simulink model "w2_warplab_buffers"  (Simulink 7.7)
settings: Solver=VariableStepDiscrete  SolverMode=SingleTasking  StartTime=0.0  StopTime=200000  RelTol=1e-3
InitFcn:
  | w2_warplab_buffers_init
StartFcn:
  | w2_warplab_buffers_init
values from neighbouring files (symbols this model uses):
  NumSamps_Rx_IQ = 2^14    (= 16384)    [w2_warplab_buffers_init.m]
  NumSamps_Rx_RSSI = 2^12    (= 4096)    [w2_warplab_buffers_init.m]
  NumSamps_Tx_IQ = 2^14    (= 16384)    [w2_warplab_buffers_init.m]
undefined symbols (not defined in the file or in its folder): gcbh, xlBlockLoadCallback, xlGetNormalizedPeriod
libraries: xbsIndex_r4 x752
(part 2 of 7)

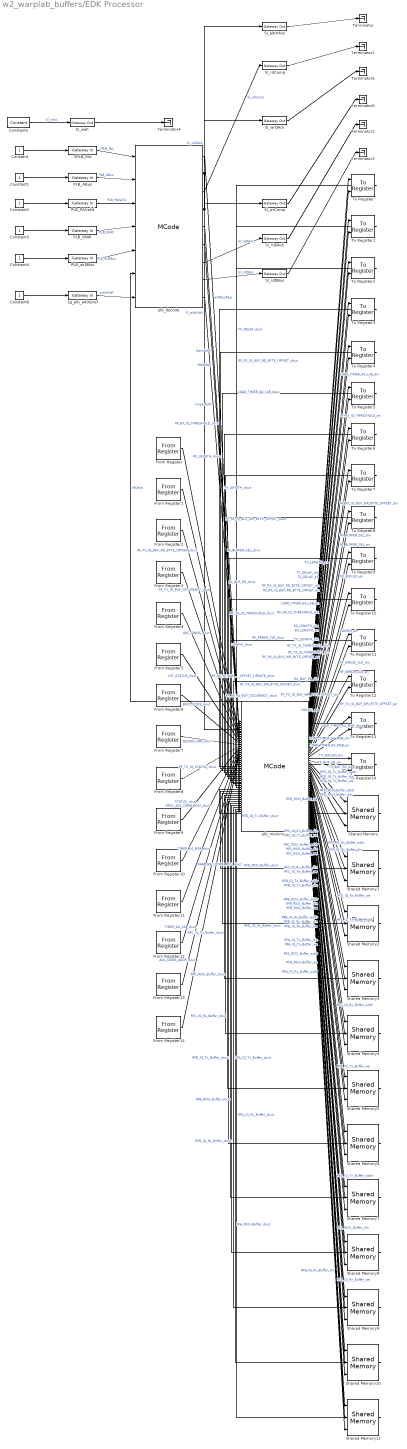
== system w2_warplab_buffers/EDK Processor ==
  Constant{,1..4,6} (6 alike) : Constant
  Constant5 : xbsIndex_r4/Constant  const=0  gui_display_data_type=Fixed-point  arith_type=Unsigned  n_bits=1  bin_pt=0  preci_type=Single  exp_width=8  frac_width=24  explicit_period=on  period=xlGetNormalizedPeriod()  equ=P=C  opselect=C  inp2=PCIN>>17  opr=+  inp1=P  carry=CIN  dbl_ovrd=off  block_type=constant
  From Register : xbsIndex_r4/From Register  shared_memory_name='RF_TX_IQ_BUF_OCCUPANCY'  init=0  period=xlGetNormalizedPeriod()  ownership=Owned and initialized elsewhere  gui_display_data_type=Fixed-point  arith_type=Unsigned  n_bits=32  bin_pt=0  preci_type=Single  dbl_ovrd=off  block_type=fromreg
      settings: AttributesFormatString=<< %<shared_memory_name> >>  infoedit="Register block that reads data to a shared memory register.  Delay of one sample period."
  From Register1 : xbsIndex_r4/From Register  shared_memory_name='RF_TX_IQ_BUF_RD_BYTE_OFFSET'  init=0  period=xlGetNormalizedPeriod()  ownership=Owned and initialized elsewhere  gui_display_data_type=Fixed-point  arith_type=Unsigned  n_bits=32  bin_pt=0  preci_type=Single  dbl_ovrd=off  block_type=fromreg
      settings: AttributesFormatString=<< %<shared_memory_name> >>  infoedit="Register block that reads data to a shared memory register.  Delay of one sample period."
  From Register10 : xbsIndex_r4/From Register  shared_memory_name='RFCD_AGC_DONE_RSSI'  init=0  period=xlGetNormalizedPeriod()  ownership=Owned and initialized elsewhere  gui_display_data_type=Fixed-point  arith_type=Unsigned  n_bits=32  bin_pt=0  preci_type=Single  dbl_ovrd=off  block_type=fromreg
      settings: AttributesFormatString=<< %<shared_memory_name> >>  infoedit="Register block that reads data to a shared memory register.  Delay of one sample period."
  From Register11 : xbsIndex_r4/From Register  shared_memory_name='RFAB_AGC_DONE_RSSI'  init=0  period=xlGetNormalizedPeriod()  ownership=Owned and initialized elsewhere  gui_display_data_type=Fixed-point  arith_type=Unsigned  n_bits=32  bin_pt=0  preci_type=Single  dbl_ovrd=off  block_type=fromreg
      settings: AttributesFormatString=<< %<shared_memory_name> >>  infoedit="Register block that reads data to a shared memory register.  Delay of one sample period."
  From Register12 : xbsIndex_r4/From Register  shared_memory_name='TIMER_64_MSB'  init=0  period=xlGetNormalizedPeriod()  ownership=Owned and initialized elsewhere  gui_display_data_type=Fixed-point  arith_type=Unsigned  n_bits=32  bin_pt=0  preci_type=Single  dbl_ovrd=off  block_type=fromreg
      settings: AttributesFormatString=<< %<shared_memory_name> >>  infoedit="Register block that reads data to a shared memory register.  Delay of one sample period."
  From Register13 : xbsIndex_r4/From Register  shared_memory_name='TIMER_64_LSB'  init=0  period=xlGetNormalizedPeriod()  ownership=Owned and initialized elsewhere  gui_display_data_type=Fixed-point  arith_type=Unsigned  n_bits=32  bin_pt=0  preci_type=Single  dbl_ovrd=off  block_type=fromreg
      settings: AttributesFormatString=<< %<shared_memory_name> >>  infoedit="Register block that reads data to a shared memory register.  Delay of one sample period."
  From Register14 : xbsIndex_r4/From Register  shared_memory_name='AGC_DONE_ADDR'  init=0  period=xlGetNormalizedPeriod()  ownership=Owned and initialized elsewhere  gui_display_data_type=Fixed-point  arith_type=Unsigned  n_bits=32  bin_pt=0  preci_type=Single  dbl_ovrd=off  block_type=fromreg
      settings: AttributesFormatString=<< %<shared_memory_name> >>  infoedit="Register block that reads data to a shared memory register.  Delay of one sample period."
  From Register2 : xbsIndex_r4/From Register  shared_memory_name='AGC_GAINS'  init=0  period=xlGetNormalizedPeriod()  ownership=Owned and initialized elsewhere  gui_display_data_type=Fixed-point  arith_type=Unsigned  n_bits=32  bin_pt=0  preci_type=Single  dbl_ovrd=off  block_type=fromreg
      settings: AttributesFormatString=<< %<shared_memory_name> >>  infoedit="Register block that reads data to a shared memory register.  Delay of one sample period."
  From Register3 : xbsIndex_r4/From Register  shared_memory_name='RF_RX_IQ_BUF_OCCUPANCY'  init=0  period=xlGetNormalizedPeriod()  ownership=Owned and initialized elsewhere  gui_display_data_type=Fixed-point  arith_type=Unsigned  n_bits=32  bin_pt=0  preci_type=Single  dbl_ovrd=off  block_type=fromreg
      settings: AttributesFormatString=<< %<shared_memory_name> >>  infoedit="Register block that reads data to a shared memory register.  Delay of one sample period."
  From Register4 : xbsIndex_r4/From Register  shared_memory_name='RF_RX_IQ_BUF_WR_BYTE_OFFSET_UPDATE'  init=0  period=xlGetNormalizedPeriod()  ownership=Owned and initialized elsewhere  gui_display_data_type=Fixed-point  arith_type=Unsigned  n_bits=32  bin_pt=0  preci_type=Single  dbl_ovrd=off  block_type=fromreg
      settings: AttributesFormatString=<< %<shared_memory_name> >>  infoedit="Register block that reads data to a shared memory register.  Delay of one sample period."
  From Register5 : xbsIndex_r4/From Register  shared_memory_name='INT_STATUS'  init=0  period=xlGetNormalizedPeriod()  ownership=Owned and initialized elsewhere  gui_display_data_type=Fixed-point  arith_type=Unsigned  n_bits=32  bin_pt=0  preci_type=Single  dbl_ovrd=off  block_type=fromreg
      settings: AttributesFormatString=<< %<shared_memory_name> >>  infoedit="Register block that reads data to a shared memory register.  Delay of one sample period."
  From Register6 : xbsIndex_r4/From Register  shared_memory_name='BUFF_SIZES'  init=0  period=xlGetNormalizedPeriod()  ownership=Owned and initialized elsewhere  gui_display_data_type=Fixed-point  arith_type=Unsigned  n_bits=32  bin_pt=0  preci_type=Single  dbl_ovrd=off  block_type=fromreg
      settings: AttributesFormatString=<< %<shared_memory_name> >>  infoedit="Register block that reads data to a shared memory register.  Delay of one sample period."
  From Register7 : xbsIndex_r4/From Register  shared_memory_name='DESIGN_VER'  init=0  period=xlGetNormalizedPeriod()  ownership=Owned and initialized elsewhere  gui_display_data_type=Fixed-point  arith_type=Unsigned  n_bits=32  bin_pt=0  preci_type=Single  dbl_ovrd=off  block_type=fromreg
      settings: AttributesFormatString=<< %<shared_memory_name> >>  infoedit="Register block that reads data to a shared memory register.  Delay of one sample period."
  From Register8 : xbsIndex_r4/From Register  shared_memory_name='RF_TX_IQ_STATUS'  init=0  period=xlGetNormalizedPeriod()  ownership=Owned and initialized elsewhere  gui_display_data_type=Fixed-point  arith_type=Unsigned  n_bits=32  bin_pt=0  preci_type=Single  dbl_ovrd=off  block_type=fromreg
      settings: AttributesFormatString=<< %<shared_memory_name> >>  infoedit="Register block that reads data to a shared memory register.  Delay of one sample period."
  From Register9 : xbsIndex_r4/From Register  shared_memory_name='STATUS'  init=0  period=xlGetNormalizedPeriod()  ownership=Owned and initialized elsewhere  gui_display_data_type=Fixed-point  arith_type=Unsigned  n_bits=32  bin_pt=0  preci_type=Single  dbl_ovrd=off  block_type=fromreg
      settings: AttributesFormatString=<< %<shared_memory_name> >>  infoedit="Register block that reads data to a shared memory register.  Delay of one sample period."
  PLB_ABus : xbsIndex_r4/Gateway In  gui_display_data_type=Fixed-point  arith_type=Unsigned  n_bits=32  bin_pt=0  preci_type=Single  exp_width=8  frac_width=24  quantization="Round  (unbiased: +/- Inf)"  overflow=Saturate  period=xlGetNormalizedPeriod()  dbl_ovrd=off  timing_constraint=None  locs_specified=off  LOCs={}  UseAsADC=off  ADCChannel='1'  inherit_from_input=off  hdl_port=on  block_type=gatewayin
      settings: sginterface={'Xilinx'=>{'jtaghwcosim'=>{'non_memory_mapped_port'=>'PLB_ABus'}},'iopad'=>{'constraint'=>'#'}}
  PLB_PAValid : xbsIndex_r4/Gateway In  gui_display_data_type=Fixed-point  arith_type=Unsigned  n_bits=1  bin_pt=0  preci_type=Single  exp_width=8  frac_width=24  quantization="Round  (unbiased: +/- Inf)"  overflow=Saturate  period=xlGetNormalizedPeriod()  dbl_ovrd=off  timing_constraint=None  locs_specified=off  LOCs={}  UseAsADC=off  ADCChannel='1'  inherit_from_input=off  hdl_port=on  block_type=gatewayin
      settings: sginterface={'Xilinx'=>{'jtaghwcosim'=>{'non_memory_mapped_port'=>'PLB_PAValid'}},'iopad'=>{'constraint'=>'#'}}
  PLB_RNW : xbsIndex_r4/Gateway In  gui_display_data_type=Fixed-point  arith_type=Unsigned  n_bits=1  bin_pt=0  preci_type=Single  exp_width=8  frac_width=24  quantization="Round  (unbiased: +/- Inf)"  overflow=Saturate  period=xlGetNormalizedPeriod()  dbl_ovrd=off  timing_constraint=None  locs_specified=off  LOCs={}  UseAsADC=off  ADCChannel='1'  inherit_from_input=off  hdl_port=on  block_type=gatewayin
      settings: sginterface={'Xilinx'=>{'jtaghwcosim'=>{'non_memory_mapped_port'=>'PLB_RNW'}},'iopad'=>{'constraint'=>'#'}}
  PLB_wrDBus : xbsIndex_r4/Gateway In  gui_display_data_type=Fixed-point  arith_type=Unsigned  n_bits=32  bin_pt=0  preci_type=Single  exp_width=8  frac_width=24  quantization="Round  (unbiased: +/- Inf)"  overflow=Saturate  period=xlGetNormalizedPeriod()  dbl_ovrd=off  timing_constraint=None  locs_specified=off  LOCs={}  UseAsADC=off  ADCChannel='1'  inherit_from_input=off  hdl_port=on  block_type=gatewayin
      settings: sginterface={'Xilinx'=>{'jtaghwcosim'=>{'non_memory_mapped_port'=>'PLB_wrDBus'}},'iopad'=>{'constraint'=>'#'}}
  SPLB_Rst : xbsIndex_r4/Gateway In  gui_display_data_type=Fixed-point  arith_type=Unsigned  n_bits=1  bin_pt=0  preci_type=Single  exp_width=8  frac_width=24  quantization="Round  (unbiased: +/- Inf)"  overflow=Saturate  period=xlGetNormalizedPeriod()  dbl_ovrd=off  timing_constraint=None  locs_specified=off  LOCs={}  UseAsADC=off  ADCChannel='1'  inherit_from_input=off  hdl_port=on  block_type=gatewayin
      settings: sginterface={'Xilinx'=>{'jtaghwcosim'=>{'non_memory_mapped_port'=>'SPLB_Rst'}},'iopad'=>{'constraint'=>'#'}}
  Shared Memory : xbsIndex_r4/Shared Memory  shared_memory_name='RFD_IQ_Tx_Buffer'  depth=16384  ownership=Owned and Initialized Elsewhere  initVector=sin(pi*(0:15)/16)  en=off  mutex=Unprotected  mode=Read and Write  write_mode=Read Before Write  time_out=0  latency=1  explicit_data_type=off  gui_display_data_type=Fixed-point  arith_type=Unsigned  n_bits=32  bin_pt=0  preci_type=Single  implementation=Block RAM  use_rpm=off  block_type=shmem
      settings: AttributesFormatString=<< %<shared_memory_name> >>
  Shared Memory1 : xbsIndex_r4/Shared Memory  shared_memory_name='RFD_RSSI_Buffer'  depth=2048  ownership=Owned and Initialized Elsewhere  initVector=sin(pi*(0:15)/16)  en=off  mutex=Unprotected  mode=Read and Write  write_mode=Read Before Write  time_out=0  latency=1  explicit_data_type=off  gui_display_data_type=Fixed-point  arith_type=Unsigned  n_bits=32  bin_pt=0  preci_type=Single  implementation=Block RAM  use_rpm=off  block_type=shmem
      settings: AttributesFormatString=<< %<shared_memory_name> >>
  Shared Memory10 : xbsIndex_r4/Shared Memory  shared_memory_name='RFA_RSSI_Buffer'  depth=2048  ownership=Owned and Initialized Elsewhere  initVector=sin(pi*(0:15)/16)  en=off  mutex=Unprotected  mode=Read and Write  write_mode=Read Before Write  time_out=0  latency=1  explicit_data_type=off  gui_display_data_type=Fixed-point  arith_type=Unsigned  n_bits=32  bin_pt=0  preci_type=Single  implementation=Block RAM  use_rpm=off  block_type=shmem
      settings: AttributesFormatString=<< %<shared_memory_name> >>
  Shared Memory11 : xbsIndex_r4/Shared Memory  shared_memory_name='RFA_IQ_Rx_Buffer'  depth=16384  ownership=Owned and Initialized Elsewhere  initVector=sin(pi*(0:15)/16)  en=off  mutex=Unprotected  mode=Read and Write  write_mode=Read Before Write  time_out=0  latency=1  explicit_data_type=off  gui_display_data_type=Fixed-point  arith_type=Unsigned  n_bits=32  bin_pt=0  preci_type=Single  implementation=Block RAM  use_rpm=off  block_type=shmem
      settings: AttributesFormatString=<< %<shared_memory_name> >>
  Shared Memory2 : xbsIndex_r4/Shared Memory  shared_memory_name='RFD_IQ_Rx_Buffer'  depth=16384  ownership=Owned and Initialized Elsewhere  initVector=sin(pi*(0:15)/16)  en=off  mutex=Unprotected  mode=Read and Write  write_mode=Read Before Write  time_out=0  latency=1  explicit_data_type=off  gui_display_data_type=Fixed-point  arith_type=Unsigned  n_bits=32  bin_pt=0  preci_type=Single  implementation=Block RAM  use_rpm=off  block_type=shmem
      settings: AttributesFormatString=<< %<shared_memory_name> >>
  Shared Memory3 : xbsIndex_r4/Shared Memory  shared_memory_name='RFC_IQ_Tx_Buffer'  depth=16384  ownership=Owned and Initialized Elsewhere  initVector=sin(pi*(0:15)/16)  en=off  mutex=Unprotected  mode=Read and Write  write_mode=Read Before Write  time_out=0  latency=1  explicit_data_type=off  gui_display_data_type=Fixed-point  arith_type=Unsigned  n_bits=32  bin_pt=0  preci_type=Single  implementation=Block RAM  use_rpm=off  block_type=shmem
      settings: AttributesFormatString=<< %<shared_memory_name> >>
  Shared Memory4 : xbsIndex_r4/Shared Memory  shared_memory_name='RFC_RSSI_Buffer'  depth=2048  ownership=Owned and Initialized Elsewhere  initVector=sin(pi*(0:15)/16)  en=off  mutex=Unprotected  mode=Read and Write  write_mode=Read Before Write  time_out=0  latency=1  explicit_data_type=off  gui_display_data_type=Fixed-point  arith_type=Unsigned  n_bits=32  bin_pt=0  preci_type=Single  implementation=Block RAM  use_rpm=off  block_type=shmem
      settings: AttributesFormatString=<< %<shared_memory_name> >>
  Shared Memory5 : xbsIndex_r4/Shared Memory  shared_memory_name='RFC_IQ_Rx_Buffer'  depth=16384  ownership=Owned and Initialized Elsewhere  initVector=sin(pi*(0:15)/16)  en=off  mutex=Unprotected  mode=Read and Write  write_mode=Read Before Write  time_out=0  latency=1  explicit_data_type=off  gui_display_data_type=Fixed-point  arith_type=Unsigned  n_bits=32  bin_pt=0  preci_type=Single  implementation=Block RAM  use_rpm=off  block_type=shmem
      settings: AttributesFormatString=<< %<shared_memory_name> >>
  Shared Memory6 : xbsIndex_r4/Shared Memory  shared_memory_name='RFB_IQ_Tx_Buffer'  depth=16384  ownership=Owned and Initialized Elsewhere  initVector=sin(pi*(0:15)/16)  en=off  mutex=Unprotected  mode=Read and Write  write_mode=Read Before Write  time_out=0  latency=1  explicit_data_type=off  gui_display_data_type=Fixed-point  arith_type=Unsigned  n_bits=32  bin_pt=0  preci_type=Single  implementation=Block RAM  use_rpm=off  block_type=shmem
      settings: AttributesFormatString=<< %<shared_memory_name> >>
  Shared Memory7 : xbsIndex_r4/Shared Memory  shared_memory_name='RFB_RSSI_Buffer'  depth=2048  ownership=Owned and Initialized Elsewhere  initVector=sin(pi*(0:15)/16)  en=off  mutex=Unprotected  mode=Read and Write  write_mode=Read Before Write  time_out=0  latency=1  explicit_data_type=off  gui_display_data_type=Fixed-point  arith_type=Unsigned  n_bits=32  bin_pt=0  preci_type=Single  implementation=Block RAM  use_rpm=off  block_type=shmem
      settings: AttributesFormatString=<< %<shared_memory_name> >>
  Shared Memory8 : xbsIndex_r4/Shared Memory  shared_memory_name='RFB_IQ_Rx_Buffer'  depth=16384  ownership=Owned and Initialized Elsewhere  initVector=sin(pi*(0:15)/16)  en=off  mutex=Unprotected  mode=Read and Write  write_mode=Read Before Write  time_out=0  latency=1  explicit_data_type=off  gui_display_data_type=Fixed-point  arith_type=Unsigned  n_bits=32  bin_pt=0  preci_type=Single  implementation=Block RAM  use_rpm=off  block_type=shmem
      settings: AttributesFormatString=<< %<shared_memory_name> >>
  Shared Memory9 : xbsIndex_r4/Shared Memory  shared_memory_name='RFA_IQ_Tx_Buffer'  depth=16384  ownership=Owned and Initialized Elsewhere  initVector=sin(pi*(0:15)/16)  en=off  mutex=Unprotected  mode=Read and Write  write_mode=Read Before Write  time_out=0  latency=1  explicit_data_type=off  gui_display_data_type=Fixed-point  arith_type=Unsigned  n_bits=32  bin_pt=0  preci_type=Single  implementation=Block RAM  use_rpm=off  block_type=shmem
      settings: AttributesFormatString=<< %<shared_memory_name> >>
  Sl_addrAck : xbsIndex_r4/Gateway Out  inherit_from_input=off  hdl_port=on  timing_constraint=None  locs_specified=off  LOCs={}  UseAsDAC=off  DACChannel='1'  block_type=gatewayout
      settings: sginterface={'Xilinx'=>{'jtaghwcosim'=>{'non_memory_mapped_port'=>'Sl_addrAck'}},'iopad'=>{'constraint'=>'#'}}
  Sl_rdComp : xbsIndex_r4/Gateway Out  inherit_from_input=off  hdl_port=on  timing_constraint=None  locs_specified=off  LOCs={}  UseAsDAC=off  DACChannel='1'  block_type=gatewayout
      settings: sginterface={'Xilinx'=>{'jtaghwcosim'=>{'non_memory_mapped_port'=>'Sl_rdComp'}},'iopad'=>{'constraint'=>'#'}}
  Sl_rdDAck : xbsIndex_r4/Gateway Out  inherit_from_input=off  hdl_port=on  timing_constraint=None  locs_specified=off  LOCs={}  UseAsDAC=off  DACChannel='1'  block_type=gatewayout
      settings: sginterface={'Xilinx'=>{'jtaghwcosim'=>{'non_memory_mapped_port'=>'Sl_rdDAck'}},'iopad'=>{'constraint'=>'#'}}
  Sl_rdDBus : xbsIndex_r4/Gateway Out  inherit_from_input=off  hdl_port=on  timing_constraint=None  locs_specified=off  LOCs={}  UseAsDAC=off  DACChannel='1'  block_type=gatewayout
      settings: sginterface={'Xilinx'=>{'jtaghwcosim'=>{'non_memory_mapped_port'=>'Sl_rdDBus'}},'iopad'=>{'constraint'=>'#'}}
  Sl_wait : xbsIndex_r4/Gateway Out  inherit_from_input=off  hdl_port=on  timing_constraint=None  locs_specified=off  LOCs={}  UseAsDAC=off  DACChannel='1'  block_type=gatewayout
      settings: sginterface={'Xilinx'=>{'jtaghwcosim'=>{'non_memory_mapped_port'=>'Sl_wait'}},'iopad'=>{'constraint'=>'#'}}
  Sl_wrComp : xbsIndex_r4/Gateway Out  inherit_from_input=off  hdl_port=on  timing_constraint=None  locs_specified=off  LOCs={}  UseAsDAC=off  DACChannel='1'  block_type=gatewayout
      settings: sginterface={'Xilinx'=>{'jtaghwcosim'=>{'non_memory_mapped_port'=>'Sl_wrComp'}},'iopad'=>{'constraint'=>'#'}}
  Sl_wrDAck : xbsIndex_r4/Gateway Out  inherit_from_input=off  hdl_port=on  timing_constraint=None  locs_specified=off  LOCs={}  UseAsDAC=off  DACChannel='1'  block_type=gatewayout
      settings: sginterface={'Xilinx'=>{'jtaghwcosim'=>{'non_memory_mapped_port'=>'Sl_wrDAck'}},'iopad'=>{'constraint'=>'#'}}
  Terminator{,1..6} (7 alike) : Terminator
  To Register : xbsIndex_r4/To Register  shared_memory_name='TX_DELAY'  init=0  ownership=Owned and initialized elsewhere  explicit_data_type=on  gui_display_data_type=Fixed-point  arith_type=Unsigned  n_bits=32  bin_pt=0  preci_type=Single  dbl_ovrd=off  block_type=toreg
      settings: AttributesFormatString=<< %<shared_memory_name> >>  infoedit="Register block that writes data to a shared memory register.  Delay of one sample period."
  To Register1 : xbsIndex_r4/To Register  shared_memory_name='RF_RX_IQ_BUF_RD_BYTE_OFFSET'  init=0  ownership=Owned and initialized elsewhere  explicit_data_type=on  gui_display_data_type=Fixed-point  arith_type=Unsigned  n_bits=32  bin_pt=0  preci_type=Single  dbl_ovrd=off  block_type=toreg
      settings: AttributesFormatString=<< %<shared_memory_name> >>  infoedit="Register block that writes data to a shared memory register.  Delay of one sample period."
  To Register10 : xbsIndex_r4/To Register  shared_memory_name='CONFIG'  init=0  ownership=Owned and initialized elsewhere  explicit_data_type=on  gui_display_data_type=Fixed-point  arith_type=Unsigned  n_bits=32  bin_pt=0  preci_type=Single  dbl_ovrd=off  block_type=toreg
      settings: AttributesFormatString=<< %<shared_memory_name> >>  infoedit="Register block that writes data to a shared memory register.  Delay of one sample period."
  To Register11 : xbsIndex_r4/To Register  shared_memory_name='RF_ERROR_CLR'  init=0  ownership=Owned and initialized elsewhere  explicit_data_type=on  gui_display_data_type=Fixed-point  arith_type=Unsigned  n_bits=9  bin_pt=0  preci_type=Single  dbl_ovrd=off  block_type=toreg
      settings: AttributesFormatString=<< %<shared_memory_name> >>  infoedit="Register block that writes data to a shared memory register.  Delay of one sample period."
  To Register12 : xbsIndex_r4/To Register  shared_memory_name='RF_TX_IQ_BUF_WR_BYTE_OFFSET'  init=0  ownership=Owned and initialized elsewhere  explicit_data_type=on  gui_display_data_type=Fixed-point  arith_type=Unsigned  n_bits=32  bin_pt=0  preci_type=Single  dbl_ovrd=off  block_type=toreg
      settings: AttributesFormatString=<< %<shared_memory_name> >>  infoedit="Register block that writes data to a shared memory register.  Delay of one sample period."
  To Register13 : xbsIndex_r4/To Register  shared_memory_name='LOAD_TIMER_64_MSB'  init=0  ownership=Owned and initialized elsewhere  explicit_data_type=on  gui_display_data_type=Fixed-point  arith_type=Unsigned  n_bits=32  bin_pt=0  preci_type=Single  dbl_ovrd=off  block_type=toreg
      settings: AttributesFormatString=<< %<shared_memory_name> >>  infoedit="Register block that writes data to a shared memory register.  Delay of one sample period."
  To Register14 : xbsIndex_r4/To Register  shared_memory_name='TX_BUF_EN'  init=0  ownership=Owned and initialized elsewhere  explicit_data_type=on  gui_display_data_type=Fixed-point  arith_type=Unsigned  n_bits=32  bin_pt=0  preci_type=Single  dbl_ovrd=off  block_type=toreg
      settings: AttributesFormatString=<< %<shared_memory_name> >>  infoedit="Register block that writes data to a shared memory register.  Delay of one sample period."
  To Register2 : xbsIndex_r4/To Register  shared_memory_name='LOAD_TIMER_64_LSB'  init=0  ownership=Owned and initialized elsewhere  explicit_data_type=on  gui_display_data_type=Fixed-point  arith_type=Unsigned  n_bits=32  bin_pt=0  preci_type=Single  dbl_ovrd=off  block_type=toreg
      settings: AttributesFormatString=<< %<shared_memory_name> >>  infoedit="Register block that writes data to a shared memory register.  Delay of one sample period."
  To Register3 : xbsIndex_r4/To Register  shared_memory_name='RF_RX_IQ_THRESHOLD'  init=0  ownership=Owned and initialized elsewhere  explicit_data_type=on  gui_display_data_type=Fixed-point  arith_type=Unsigned  n_bits=32  bin_pt=0  preci_type=Single  dbl_ovrd=off  block_type=toreg
      settings: AttributesFormatString=<< %<shared_memory_name> >>  infoedit="Register block that writes data to a shared memory register.  Delay of one sample period."
  To Register4 : xbsIndex_r4/To Register  shared_memory_name='RX_LENGTH'  init=0  ownership=Owned and initialized elsewhere  explicit_data_type=on  gui_display_data_type=Fixed-point  arith_type=Unsigned  n_bits=32  bin_pt=0  preci_type=Single  dbl_ovrd=off  block_type=toreg
      settings: AttributesFormatString=<< %<shared_memory_name> >>  infoedit="Register block that writes data to a shared memory register.  Delay of one sample period."
  To Register5 : xbsIndex_r4/To Register  shared_memory_name='TX_LENGTH'  init=0  ownership=Owned and initialized elsewhere  explicit_data_type=on  gui_display_data_type=Fixed-point  arith_type=Unsigned  n_bits=32  bin_pt=0  preci_type=Single  dbl_ovrd=off  block_type=toreg
      settings: AttributesFormatString=<< %<shared_memory_name> >>  infoedit="Register block that writes data to a shared memory register.  Delay of one sample period."
  To Register6 : xbsIndex_r4/To Register  shared_memory_name='RF_RX_IQ_BUF_WR_BYTE_OFFSET'  init=0  ownership=Owned and initialized elsewhere  explicit_data_type=on  gui_display_data_type=Fixed-point  arith_type=Unsigned  n_bits=32  bin_pt=0  preci_type=Single  dbl_ovrd=off  block_type=toreg
      settings: AttributesFormatString=<< %<shared_memory_name> >>  infoedit="Register block that writes data to a shared memory register.  Delay of one sample period."
  To Register7 : xbsIndex_r4/To Register  shared_memory_name='RF_BUFFER_SEL'  init=0  ownership=Owned and initialized elsewhere  explicit_data_type=on  gui_display_data_type=Fixed-point  arith_type=Unsigned  n_bits=32  bin_pt=0  preci_type=Single  dbl_ovrd=off  block_type=toreg
      settings: AttributesFormatString=<< %<shared_memory_name> >>  infoedit="Register block that writes data to a shared memory register.  Delay of one sample period."
  To Register8 : xbsIndex_r4/To Register  shared_memory_name='RX_BUF_EN'  init=0  ownership=Owned and initialized elsewhere  explicit_data_type=on  gui_display_data_type=Fixed-point  arith_type=Unsigned  n_bits=32  bin_pt=0  preci_type=Single  dbl_ovrd=off  block_type=toreg
      settings: AttributesFormatString=<< %<shared_memory_name> >>  infoedit="Register block that writes data to a shared memory register.  Delay of one sample period."
  To Register9 : xbsIndex_r4/To Register  shared_memory_name='RF_TX_IQ_THRESHOLD'  init=0  ownership=Owned and initialized elsewhere  explicit_data_type=on  gui_display_data_type=Fixed-point  arith_type=Unsigned  n_bits=32  bin_pt=0  preci_type=Single  dbl_ovrd=off  block_type=toreg
      settings: AttributesFormatString=<< %<shared_memory_name> >>  infoedit="Register block that writes data to a shared memory register.  Delay of one sample period."
  plb_decode : xbsIndex_r4/MCode  mfname=xlmax  explicit_period=off  period=1  dbl_ovrd=off  enable_stdout=off  enable_debug=off  mfilecontent=|  suppress_output=on  defparams={}  hide_port_list={}  block_type=mcode
      | function [wrDBusReg, addrAck, rdComp, wrDAck, bankAddr, RNWReg, rdDAck, rdDBus, linearAddr] = plb_bus_decode(plbRst, plbABus, plbPAValid, plbRNW, plbWrDBus, rdData, addrPref)
      | 
      | % constant variables (TODO: should pass from outside)
      | ADDRPREF_LEN = 10;
      | BANKADDR_LEN = 2;
      | LINEARADDR_LEN = 18;
      | ABUS_LEN = 32;
      | DBUS_LEN = 32;
      | 
      | % declare and initialize persistent variables
      | % register input bus signals
      | persistent plbRstReg_, plbRstReg_ = xl_state(0, {xlBoolean});
      | persistent plbABusReg_, plbABusReg_ = xl_state(0, {xlUnsigned, ABUS_LEN, 0});
      | persistent plbPAValidReg_, plbPAValidReg_ = xl_state(0, {xlBoolean});
      | persistent plbRNWReg_, plbRNWReg_ = xl_state(0, {xlUnsigned, 1, 0});
      | persistent plbWrDBusReg_, plbWrDBusReg_ = xl_state(0, {xlUnsigned, DBUS_LEN, 0});
      | 
      | % ===== rest of the outputs =====
      | 
      | bankAddr   = xl_slice(plbABusReg_, 2+BANKADDR_LEN+LINEARADDR_LEN-1, 2+LINEARADDR_LEN);
      | linearAddr = xl_slice(plbABusReg_, 2+LINEARADDR_LEN-1, 2);
      | RNWReg = plbRNWReg_;
      | wrDBusReg = plbWrDBusReg_;
      | 
      | % ===== p_select =====
      | 
      | % register PAValid
      | persistent aValidReg, aValidReg = xl_state(0, {xlBoolean});
      | aValidReg = plbPAValidReg_;
      | 
      | % extract and register the address prefix
      | addrPref_in = xl_slice(plbABusReg_, xl_nbits(plbABusReg_)-1, xl_nbits(plbABusReg_)-ADDRPREF_LEN);
      | if addrPref_in == addrPref
      |     ps1 = true;
      | else 
      |     ps1 = false;
      | end 
      | 
      | persistent ps1Reg, ps1Reg = xl_state(0, ps1);
      | ps1Reg = ps1;
      | 
      | ps = xl_and(ps1Reg, aValidReg);
      | 
      | % ===== addrAck =====
      | 
      | % register ps
      | persistent psReg, psReg = xl_state(0, ps);
      | 
      | addrAck = xfix({xlUnsigned, 1, 0}, xl_and(xl_not(plbRstReg_), ps, xl_not(psReg)));
      | 
      | psReg = ps;
      | 
      | % ===== rdComp, rd/wr DAck =====
      |  
      | rdComp1 = xfix({xlUnsigned, 1, 0}, xl_and(addrAck, RNWReg));
      | 
      | NUM_rdCompDelay = 3;
      | persistent rdCompDelay, rdCompDelay = xl_state(zeros(1, NUM_rdCompDelay), rdComp1, NUM_rdCompDelay);
      | rdComp2 = rdCompDelay.back;
      | rdCompDelay.push_front_pop_back(rdComp1);
      | 
      | persistent rdCompReg, rdCompReg = xl_state(0, rdComp1);
      | rdComp = rdCompReg;
      | rdCompReg = rdComp2;
      | 
      | persistent rdDAckReg, rdDAckReg = xl_state(0, rdComp1);
      | rdDAck = rdDAckReg;
      | rdDAckReg = rdComp;
      | 
      | persistent wrDAckReg, wrDAckReg = xl_state(0, addrAck);
      | wrDAck = wrDAckReg;
      | wrDAckReg = xl_and(addrAck, xl_not(RNWReg));
      | 
      | % ===== rdDBus =====
      | 
      | rdSel = xl_or(rdComp2, rdComp);
      | 
      | if rdSel == 1
      |     rdDBus1 = rdData;
      | else
      |     rdDBus1 = 0;
      | end % if
      | 
      | persistent rdDBusReg, rdDBusReg = xl_state(0, rdDBus1);
      | rdDBus = rdDBusReg;
      | rdDBusReg = rdDBus1;
      | 
      | % rdDBus = xl_concat(rdDBus32, rdDBus32);
      | % rdDBus = rdDBus32;
      | 
      | % ===== update the persistent variables =====
      | 
      | plbRstReg_ = plbRst;
      | plbABusReg_ = plbABus;
      | plbPAValidReg_ = plbPAValid;
      | plbRNWReg_ = plbRNW;
      | plbWrDBusReg_ = xl_slice(plbWrDBus, DBUS_LEN-1, 0);
  plb_memmap : xbsIndex_r4/MCode  mfname=xlmax  explicit_period=off  period=1  dbl_ovrd=off  enable_stdout=off  enable_debug=off  mfilecontent=|  suppress_output=on  defparams={}  hide_port_list={}  block_type=mcode
      | function [read_bank_out, sm_TX_DELAY_din, sm_TX_DELAY_en, sm_RF_RX_IQ_BUF_RD_BYTE_OFFSET_din, sm_RF_RX_IQ_BUF_RD_BYTE_OFFSET_en, sm_LOAD_TIMER_64_LSB_din, sm_LOAD_TIMER_64_LSB_en, sm_RF_RX_IQ_THRESHOLD_din, sm_RF_RX_IQ_THRESHOLD_en, sm_RX_LENGTH_din, sm_RX_LENGTH_en, sm_TX_LENGTH_din, sm_TX_LENGTH_en, sm_RF_RX_IQ_BUF_WR_BYTE_OFFSET_din, sm_RF_RX_IQ_BUF_WR_BYTE_OFFSET_en, sm_RF_BUFFER_SEL_din, sm_RF_BUFFER_SEL_en, sm_RX_BUF_EN_din, sm_RX_BUF_EN_en, sm_RF_TX_IQ_THRESHOLD_din, sm_RF_TX_IQ_THRESHOLD_en, sm_CONFIG_din, sm_CONFIG_en, sm_RF_ERROR_CLR_din, sm_RF_ERROR_CLR_en, sm_RF_TX_IQ_BUF_WR_BYTE_OFFSET_din, sm_RF_TX_IQ_BUF_WR_BYTE_OFFSET_en, sm_LOAD_TIMER_64_MSB_din, sm_LOAD_TIMER_64_MSB_en, sm_TX_BUF_EN_din, sm_TX_BUF_EN_en, sm_RFD_IQ_Tx_Buffer_addr, sm_RFD_IQ_Tx_Buffer_din, sm_RFD_IQ_Tx_Buffer_we, sm_RFD_RSSI_Buffer_addr, sm_RFD_RSSI_Buffer_din, sm_RFD_RSSI_Buffer_we, sm_RFD_IQ_Rx_Buffer_addr, sm_RFD_IQ_Rx_Buffer_din, sm_RFD_IQ_Rx_Buffer_we, sm_RFC_IQ_Tx_Buffer_addr, sm_RFC_IQ_Tx_Buffer_din, sm_RFC_IQ_Tx_Buffer_we, sm_RFC_RSSI_Buffer_addr, sm_RFC_RSSI_Buffer_din, sm_RFC_RSSI_Buffer_we, sm_RFC_IQ_Rx_Buffer_addr, sm_RFC_IQ_Rx_Buffer_din, sm_RFC_IQ_Rx_Buffer_we, sm_RFB_IQ_Tx_Buffer_addr, sm_RFB_IQ_Tx_Buffer_din, sm_RFB_IQ_Tx_Buffer_we, sm_RFB_RSSI_Buffer_addr, sm_RFB_RSSI_Buffer_din, sm_RFB_RSSI_Buffer_we, sm_RFB_IQ_Rx_Buffer_addr, sm_RFB_IQ_Rx_Buffer_din, sm_RFB_IQ_Rx_Buffer_we, sm_RFA_IQ_Tx_Buffer_addr, sm_RFA_IQ_Tx_Buffer_din, sm_RFA_IQ_Tx_Buffer_we, sm_RFA_RSSI_Buffer_addr, sm_RFA_RSSI_Buffer_din, sm_RFA_RSSI_Buffer_we, sm_RFA_IQ_Rx_Buffer_addr, sm_RFA_IQ_Rx_Buffer_din, sm_RFA_IQ_Rx_Buffer_we] = plb_memmap(wrDBus, bankAddr, linearAddr, RNWReg, addrAck, sm_RF_TX_IQ_BUF_OCCUPANCY, sm_RF_TX_IQ_BUF_RD_BYTE_OFFSET, sm_AGC_GAINS, sm_RF_RX_IQ_BUF_OCCUPANCY, sm_RF_RX_IQ_BUF_WR_BYTE_OFFSET_UPDATE, sm_INT_STATUS, sm_BUFF_SIZES, sm_DESIGN_VER, sm_RF_TX_IQ_STATUS, sm_STATUS, sm_RFCD_AGC_DONE_RSSI, sm_RFAB_AGC_DONE_RSSI, sm_TIMER_64_MSB, sm_TIMER_64_LSB, sm_AGC_DONE_ADDR, sm_TX_DELAY, sm_RF_RX_IQ_BUF_RD_BYTE_OFFSET, sm_LOAD_TIMER_64_LSB, sm_RF_RX_IQ_THRESHOLD, sm_RX_LENGTH, sm_TX_LENGTH, sm_RF_RX_IQ_BUF_WR_BYTE_OFFSET, sm_RF_BUFFER_SEL, sm_RX_BUF_EN, sm_RF_TX_IQ_THRESHOLD, sm_CONFIG, sm_RF_ERROR_CLR, sm_RF_TX_IQ_BUF_WR_BYTE_OFFSET, sm_LOAD_TIMER_64_MSB, sm_TX_BUF_EN, sm_RFD_IQ_Tx_Buffer, sm_RFD_RSSI_Buffer, sm_RFD_IQ_Rx_Buffer, sm_RFC_IQ_Tx_Buffer, sm_RFC_RSSI_Buffer, sm_RFC_IQ_Rx_Buffer, sm_RFB_IQ_Tx_Buffer, sm_RFB_RSSI_Buffer, sm_RFB_IQ_Rx_Buffer, sm_RFA_IQ_Tx_Buffer, sm_RFA_RSSI_Buffer, sm_RFA_IQ_Rx_Buffer)
      | 
      | 
      | % connvert the input data to UFix_32_0 (the bus data type)
      | % 'From Register' blocks
      | % sm_RF_TX_IQ_BUF_OCCUPANCY_bus = xfix({xlUnsigned, 32, 0}, 0);
      | sm_RF_TX_IQ_BUF_OCCUPANCY_bus = xl_force(sm_RF_TX_IQ_BUF_OCCUPANCY, xlUnsigned, 0);
      | 
      | % sm_RF_TX_IQ_BUF_RD_BYTE_OFFSET_bus = xfix({xlUnsigned, 32, 0}, 0);
      | sm_RF_TX_IQ_BUF_RD_BYTE_OFFSET_bus = xl_force(sm_RF_TX_IQ_BUF_RD_BYTE_OFFSET, xlUnsigned, 0);
      | 
      | % sm_AGC_GAINS_bus = xfix({xlUnsigned, 32, 0}, 0);
      | sm_AGC_GAINS_bus = xl_force(sm_AGC_GAINS, xlUnsigned, 0);
      | 
      | % sm_RF_RX_IQ_BUF_OCCUPANCY_bus = xfix({xlUnsigned, 32, 0}, 0);
      | sm_RF_RX_IQ_BUF_OCCUPANCY_bus = xl_force(sm_RF_RX_IQ_BUF_OCCUPANCY, xlUnsigned, 0);
      | 
      | % sm_RF_RX_IQ_BUF_WR_BYTE_OFFSET_UPDATE_bus = xfix({xlUnsigned, 32, 0}, 0);
      | sm_RF_RX_IQ_BUF_WR_BYTE_OFFSET_UPDATE_bus = xl_force(sm_RF_RX_IQ_BUF_WR_BYTE_OFFSET_UPDATE, xlUnsigned, 0);
      | 
      | % sm_INT_STATUS_bus = xfix({xlUnsigned, 32, 0}, 0);
      | sm_INT_STATUS_bus = xl_force(sm_INT_STATUS, xlUnsigned, 0);
      | 
      | % sm_BUFF_SIZES_bus = xfix({xlUnsigned, 32, 0}, 0);
      | sm_BUFF_SIZES_bus = xl_force(sm_BUFF_SIZES, xlUnsigned, 0);
      | 
      | % sm_DESIGN_VER_bus = xfix({xlUnsigned, 32, 0}, 0);
      | sm_DESIGN_VER_bus = xl_force(sm_DESIGN_VER, xlUnsigned, 0);
      | 
      | % sm_RF_TX_IQ_STATUS_bus = xfix({xlUnsigned, 32, 0}, 0);
      | sm_RF_TX_IQ_STATUS_bus = xl_force(sm_RF_TX_IQ_STATUS, xlUnsigned, 0);
      | 
      | % sm_STATUS_bus = xfix({xlUnsigned, 32, 0}, 0);
      | sm_STATUS_bus = xl_force(sm_STATUS, xlUnsigned, 0);
      | 
      | % sm_RFCD_AGC_DONE_RSSI_bus = xfix({xlUnsigned, 32, 0}, 0);
      | sm_RFCD_AGC_DONE_RSSI_bus = xl_force(sm_RFCD_AGC_DONE_RSSI, xlUnsigned, 0);
      | 
      | % sm_RFAB_AGC_DONE_RSSI_bus = xfix({xlUnsigned, 32, 0}, 0);
      | sm_RFAB_AGC_DONE_RSSI_bus = xl_force(sm_RFAB_AGC_DONE_RSSI, xlUnsigned, 0);
      | 
      | % sm_TIMER_64_MSB_bus = xfix({xlUnsigned, 32, 0}, 0);
      | sm_TIMER_64_MSB_bus = xl_force(sm_TIMER_64_MSB, xlUnsigned, 0);
      | 
      | % sm_TIMER_64_LSB_bus = xfix({xlUnsigned, 32, 0}, 0);
      | sm_TIMER_64_LSB_bus = xl_force(sm_TIMER_64_LSB, xlUnsigned, 0);
      | 
      | % sm_AGC_DONE_ADDR_bus = xfix({xlUnsigned, 32, 0}, 0);
      | sm_AGC_DONE_ADDR_bus = xl_force(sm_AGC_DONE_ADDR, xlUnsigned, 0);
      | 
      | % 'To Register' blocks
      | 
      | % sm_TX_DELAY_dout = xfix({xlUnsigned, 32, 0}, 0);
      | sm_TX_DELAY_dout = xl_force(sm_TX_DELAY, xlUnsigned, 0);
      | 
      | % sm_RF_RX_IQ_BUF_RD_BYTE_OFFSET_dout = xfix({xlUnsigned, 32, 0}, 0);
      | sm_RF_RX_IQ_BUF_RD_BYTE_OFFSET_dout = xl_force(sm_RF_RX_IQ_BUF_RD_BYTE_OFFSET, xlUnsigned, 0);
      | 
      | % sm_LOAD_TIMER_64_LSB_dout = xfix({xlUnsigned, 32, 0}, 0);
      | sm_LOAD_TIMER_64_LSB_dout = xl_force(sm_LOAD_TIMER_64_LSB, xlUnsigned, 0);
      | 
      | % sm_RF_RX_IQ_THRESHOLD_dout = xfix({xlUnsigned, 32, 0}, 0);
      | sm_RF_RX_IQ_THRESHOLD_dout = xl_force(sm_RF_RX_IQ_THRESHOLD, xlUnsigned, 0);
      | 
      | % sm_RX_LENGTH_dout = xfix({xlUnsigned, 32, 0}, 0);
      | sm_RX_LENGTH_dout = xl_force(sm_RX_LENGTH, xlUnsigned, 0);
      | 
      | % sm_TX_LENGTH_dout = xfix({xlUnsigned, 32, 0}, 0);
      | sm_TX_LENGTH_dout = xl_force(sm_TX_LENGTH, xlUnsigned, 0);
      | 
      | % sm_RF_RX_IQ_BUF_WR_BYTE_OFFSET_dout = xfix({xlUnsigned, 32, 0}, 0);
      | sm_RF_RX_IQ_BUF_WR_BYTE_OFFSET_dout = xl_force(sm_RF_RX_IQ_BUF_WR_BYTE_OFFSET, xlUnsigned, 0);
      | 
      | % sm_RF_BUFFER_SEL_dout = xfix({xlUnsigned, 32, 0}, 0);
      | sm_RF_BUFFER_SEL_dout = xl_force(sm_RF_BUFFER_SEL, xlUnsigned, 0);
      | 
      | % sm_RX_BUF_EN_dout = xfix({xlUnsigned, 32, 0}, 0);
      | sm_RX_BUF_EN_dout = xl_force(sm_RX_BUF_EN, xlUnsigned, 0);
      | 
      | % sm_RF_TX_IQ_THRESHOLD_dout = xfix({xlUnsigned, 32, 0}, 0);
      | sm_RF_TX_IQ_THRESHOLD_dout = xl_force(sm_RF_TX_IQ_THRESHOLD, xlUnsigned, 0);
      | 
      | % sm_CONFIG_dout = xfix({xlUnsigned, 32, 0}, 0);
      | sm_CONFIG_dout = xl_force(sm_CONFIG, xlUnsigned, 0);
      | 
      | % sm_RF_ERROR_CLR_dout = xfix({xlUnsigned, 32, 0}, 0);
      | sm_RF_ERROR_CLR_dout = xl_force(sm_RF_ERROR_CLR, xlUnsigned, 0);
      | 
      | % sm_RF_TX_IQ_BUF_WR_BYTE_OFFSET_dout = xfix({xlUnsigned, 32, 0}, 0);
      | sm_RF_TX_IQ_BUF_WR_BYTE_OFFSET_dout = xl_force(sm_RF_TX_IQ_BUF_WR_BYTE_OFFSET, xlUnsigned, 0);
      | 
      | % sm_LOAD_TIMER_64_MSB_dout = xfix({xlUnsigned, 32, 0}, 0);
      | sm_LOAD_TIMER_64_MSB_dout = xl_force(sm_LOAD_TIMER_64_MSB, xlUnsigned, 0);
      | 
      | % sm_TX_BUF_EN_dout = xfix({xlUnsigned, 32, 0}, 0);
      | sm_TX_BUF_EN_dout = xl_force(sm_TX_BUF_EN, xlUnsigned, 0);
      | 
      | 
      | % 'From FIFO' blocks
      | % 'To FIFO' blocks
      | % 'Shared Memory' blocks
      | % RFD_IQ_Tx_Buffer_bus = xfix({xlUnsigned, 32, 0}, 0);
      | sm_RFD_IQ_Tx_Buffer_bus = xl_force(sm_RFD_IQ_Tx_Buffer, xlUnsigned, 0);
      | 
      | % RFD_RSSI_Buffer_bus = xfix({xlUnsigned, 32, 0}, 0);
      | sm_RFD_RSSI_Buffer_bus = xl_force(sm_RFD_RSSI_Buffer, xlUnsigned, 0);
      | 
      | % RFD_IQ_Rx_Buffer_bus = xfix({xlUnsigned, 32, 0}, 0);
      | sm_RFD_IQ_Rx_Buffer_bus = xl_force(sm_RFD_IQ_Rx_Buffer, xlUnsigned, 0);
      | 
      | % RFC_IQ_Tx_Buffer_bus = xfix({xlUnsigned, 32, 0}, 0);
      | sm_RFC_IQ_Tx_Buffer_bus = xl_force(sm_RFC_IQ_Tx_Buffer, xlUnsigned, 0);
      | 
      | % RFC_RSSI_Buffer_bus = xfix({xlUnsigned, 32, 0}, 0);
      | sm_RFC_RSSI_Buffer_bus = xl_force(sm_RFC_RSSI_Buffer, xlUnsigned, 0);
      | 
      | % RFC_IQ_Rx_Buffer_bus = xfix({xlUnsigned, 32, 0}, 0);
      | sm_RFC_IQ_Rx_Buffer_bus = xl_force(sm_RFC_IQ_Rx_Buffer, xlUnsigned, 0);
      | 
      | % RFB_IQ_Tx_Buffer_bus = xfix({xlUnsigned, 32, 0}, 0);
      | sm_RFB_IQ_Tx_Buffer_bus = xl_force(sm_RFB_IQ_Tx_Buffer, xlUnsigned, 0);
      | 
      | % RFB_RSSI_Buffer_bus = xfix({xlUnsigned, 32, 0}, 0);
      | sm_RFB_RSSI_Buffer_bus = xl_force(sm_RFB_RSSI_Buffer, xlUnsigned, 0);
      | 
      | % RFB_IQ_Rx_Buffer_bus = xfix({xlUnsigned, 32, 0}, 0);
      | sm_RFB_IQ_Rx_Buffer_bus = xl_force(sm_RFB_IQ_Rx_Buffer, xlUnsigned, 0);
      | 
      | % RFA_IQ_Tx_Buffer_bus = xfix({xlUnsigned, 32, 0}, 0);
      | sm_RFA_IQ_Tx_Buffer_bus = xl_force(sm_RFA_IQ_Tx_Buffer, xlUnsigned, 0);
      | 
      | % RFA_RSSI_Buffer_bus = xfix({xlUnsigned, 32, 0}, 0);
      | sm_RFA_RSSI_Buffer_bus = xl_force(sm_RFA_RSSI_Buffer, xlUnsigned, 0);
      | 
      | % RFA_IQ_Rx_Buffer_bus = xfix({xlUnsigned, 32, 0}, 0);
      | sm_RFA_IQ_Rx_Buffer_bus = xl_force(sm_RFA_IQ_Rx_Buffer, xlUnsigned, 0);
      | 
      | 
      | % 'dout' ports of 'From Register' blocks
      | 
      | % registered register mux output
      | persistent reg_bank_out_reg; reg_bank_out_reg = xl_state(0, {xlUnsigned, 32, 0});
      | reg_bank_out = reg_bank_out_reg;
      | 
      | if linearAddr == 15
      |     reg_bank_out_reg = sm_RF_TX_IQ_BUF_OCCUPANCY_bus;
      | elseif linearAddr == 16
      |     reg_bank_out_reg = sm_RF_TX_IQ_BUF_RD_BYTE_OFFSET_bus;
      | elseif linearAddr == 17
      |     reg_bank_out_reg = sm_AGC_GAINS_bus;
      | elseif linearAddr == 18
      |     reg_bank_out_reg = sm_RF_RX_IQ_BUF_OCCUPANCY_bus;
      | elseif linearAddr == 19
      |     reg_bank_out_reg = sm_RF_RX_IQ_BUF_WR_BYTE_OFFSET_UPDATE_bus;
      | elseif linearAddr == 20
      |     reg_bank_out_reg = sm_INT_STATUS_bus;
      | elseif linearAddr == 21
      |     reg_bank_out_reg = sm_BUFF_SIZES_bus;
      | elseif linearAddr == 22
      |     reg_bank_out_reg = sm_DESIGN_VER_bus;
      | elseif linearAddr == 23
      |     reg_bank_out_reg = sm_RF_TX_IQ_STATUS_bus;
      | elseif linearAddr == 24
      |     reg_bank_out_reg = sm_STATUS_bus;
      | elseif linearAddr == 25
      |     reg_bank_out_reg = sm_RFCD_AGC_DONE_RSSI_bus;
      | elseif linearAddr == 26
      |     reg_bank_out_reg = sm_RFAB_AGC_DONE_RSSI_bus;
      | elseif linearAddr == 27
      |     reg_bank_out_reg = sm_TIMER_64_MSB_bus;
      | elseif linearAddr == 28
      |     reg_bank_out_reg = sm_TIMER_64_LSB_bus;
      | elseif linearAddr == 29
      |     reg_bank_out_reg = sm_AGC_DONE_ADDR_bus;
      | elseif linearAddr == 0
      |     reg_bank_out_reg = sm_TX_DELAY_dout;
      | elseif linearAddr == 1
      |     reg_bank_out_reg = sm_RF_RX_IQ_BUF_RD_BYTE_OFFSET_dout;
      | elseif linearAddr == 2
      |     reg_bank_out_reg = sm_LOAD_TIMER_64_LSB_dout;
      | elseif linearAddr == 3
      |     reg_bank_out_reg = sm_RF_RX_IQ_THRESHOLD_dout;
      | elseif linearAddr == 4
      |     reg_bank_out_reg = sm_RX_LENGTH_dout;
      | elseif linearAddr == 5
      |     reg_bank_out_reg = sm_TX_LENGTH_dout;
      | elseif linearAddr == 6
      |     reg_bank_out_reg = sm_RF_RX_IQ_BUF_WR_BYTE_OFFSET_dout;
      | elseif linearAddr == 7
      |     reg_bank_out_reg = sm_RF_BUFFER_SEL_dout;
      | elseif linearAddr == 8
      |     reg_bank_out_reg = sm_RX_BUF_EN_dout;
      | elseif linearAddr == 9
      |     reg_bank_out_reg = sm_RF_TX_IQ_THRESHOLD_dout;
      | elseif linearAddr == 10
      |     reg_bank_out_reg = sm_CONFIG_dout;
      | elseif linearAddr == 11
      |     reg_bank_out_reg = sm_RF_ERROR_CLR_dout;
      | elseif linearAddr == 12
      |     reg_bank_out_reg = sm_RF_TX_IQ_BUF_WR_BYTE_OFFSET_dout;
      | elseif linearAddr == 13
      |     reg_bank_out_reg = sm_LOAD_TIMER_64_MSB_dout;
      | elseif linearAddr == 14
      |     reg_bank_out_reg = sm_TX_BUF_EN_dout;
      | 
      | end
      | 
      | 
      | % 'From FIFO' and 'To FIFO' blocks
      | 
      | 
      | 
      | 
      | 
      | opCode = xl_concat(addrAck, RNWReg, bankAddr, linearAddr);
      | 
      | % 'Shared Memory' blocks
      | 
      | sm_RFD_IQ_Tx_Buffer_sel_value = xl_concat(xl_slice(linearAddr, ...
      |                                         xl_nbits(linearAddr) - 1, ...
      |                                         14) ...
      |                                     );
      | if sm_RFD_IQ_Tx_Buffer_sel_value == xfix({xlUnsigned, ...
      |                                         xl_nbits(linearAddr) - 14, ...
      |                                         0}, ...
      |                                         0);
      |     sm_RFD_IQ_Tx_Buffer_sel = true;
      | else
      |     sm_RFD_IQ_Tx_Buffer_sel = false;
      | end
      | sm_RFD_RSSI_Buffer_sel_value = xl_concat(xl_slice(linearAddr, ...
      |                                         xl_nbits(linearAddr) - 1, ...
      |                                         11) ...
      |                                     );
      | if sm_RFD_RSSI_Buffer_sel_value == xfix({xlUnsigned, ...
      |                                         xl_nbits(linearAddr) - 11, ...
      |                                         0}, ...
      |                                         64);
      |     sm_RFD_RSSI_Buffer_sel = true;
      | else
      |     sm_RFD_RSSI_Buffer_sel = false;
      | end
      | sm_RFD_IQ_Rx_Buffer_sel_value = xl_concat(xl_slice(linearAddr, ...
      |                                         xl_nbits(linearAddr) - 1, ...
      |                                         14) ...
      |                                     );
      | if sm_RFD_IQ_Rx_Buffer_sel_value == xfix({xlUnsigned, ...
      |                                         xl_nbits(linearAddr) - 14, ...
      |                                         0}, ...
      |                                         1);
      |     sm_RFD_IQ_Rx_Buffer_sel = true;
      | else
      |     sm_RFD_IQ_Rx_Buffer_sel = false;
      | end
      | sm_RFC_IQ_Tx_Buffer_sel_value = xl_concat(xl_slice(linearAddr, ...
      |                                         xl_nbits(linearAddr) - 1, ...
      |                                         14) ...
      |                                     );
      | if sm_RFC_IQ_Tx_Buffer_sel_value == xfix({xlUnsigned, ...
      |                                         xl_nbits(linearAddr) - 14, ...
      |                                         0}, ...
      |                                         2);
      |     sm_RFC_IQ_Tx_Buffer_sel = true;
      | else
      |     sm_RFC_IQ_Tx_Buffer_sel = false;
      | end
      | sm_RFC_RSSI_Buffer_sel_value = xl_concat(xl_slice(linearAddr, ...
      |                                         xl_nbits(linearAddr) - 1, ...
      |                                         11) ...
      |                                     );
      | if sm_RFC_RSSI_Buffer_sel_value == xfix({xlUnsigned, ...
      |                                         xl_nbits(linearAddr) - 11, ...
      |                                         0}, ...
      |                                         65);
      |     sm_RFC_RSSI_Buffer_sel = true;
      | else
      |     sm_RFC_RSSI_Buffer_sel = false;
      | end
      | sm_RFC_IQ_Rx_Buffer_sel_value = xl_concat(xl_slice(linearAddr, ...
      |                                         xl_nbits(linearAddr) - 1, ...
      |                                         14) ...
      |                                     );
      | if sm_RFC_IQ_Rx_Buffer_sel_value == xfix({xlUnsigned, ...
      |                                         xl_nbits(linearAddr) - 14, ...
      |                                         0}, ...
      |                                         3);
      |     sm_RFC_IQ_Rx_Buffer_sel = true;
      | else
      |     sm_RFC_IQ_Rx_Buffer_sel = false;
      | end
      | sm_RFB_IQ_Tx_Buffer_sel_value = xl_concat(xl_slice(linearAddr, ...
      |                                         xl_nbits(linearAddr) - 1, ...
      |                                         14) ...
      |                                     );
      | if sm_RFB_IQ_Tx_Buffer_sel_value == xfix({xlUnsigned, ...
      |                                         xl_nbits(linearAddr) - 14, ...
      |                                         0}, ...
      |                                         4);
      |     sm_RFB_IQ_Tx_Buffer_sel = true;
      | else
      |     sm_RFB_IQ_Tx_Buffer_sel = false;
      | end
      | sm_RFB_RSSI_Buffer_sel_value = xl_concat(xl_slice(linearAddr, ...
      |                                         xl_nbits(linearAddr) - 1, ...
      |                                         11) ...
      |                                     );
      | if sm_RFB_RSSI_Buffer_sel_value == xfix({xlUnsigned, ...
      |                                         xl_nbits(linearAddr) - 11, ...
      |                                         0}, ...
      |                                         66);
      |     sm_RFB_RSSI_Buffer_sel = true;
      | else
      |     sm_RFB_RSSI_Buffer_sel = false;
      | end
      | sm_RFB_IQ_Rx_Buffer_sel_value = xl_concat(xl_slice(linearAddr, ...
      |                                         xl_nbits(linearAddr) - 1, ...
      |                                         14) ...
      |                                     );
      | if sm_RFB_IQ_Rx_Buffer_sel_value == xfix({xlUnsigned, ...
      |                                         xl_nbits(linearAddr) - 14, ...
      |                                         0}, ...
      |                                         5);
      |     sm_RFB_IQ_Rx_Buffer_sel = true;
      | else
      |     sm_RFB_IQ_Rx_Buffer_sel = false;
      | end
      | sm_RFA_IQ_Tx_Buffer_sel_value = xl_concat(xl_slice(linearAddr, ...
      |                                         xl_nbits(linearAddr) - 1, ...
      |                                         14) ...
      |                                     );
      | if sm_RFA_IQ_Tx_Buffer_sel_value == xfix({xlUnsigned, ...
      |                                         xl_nbits(linearAddr) - 14, ...
      |                                         0}, ...
      |                                         6);
      |     sm_RFA_IQ_Tx_Buffer_sel = true;
      | else
      |     sm_RFA_IQ_Tx_Buffer_sel = false;
      | end
      | sm_RFA_RSSI_Buffer_sel_value = xl_concat(xl_slice(linearAddr, ...
      |                                         xl_nbits(linearAddr) - 1, ...
      |                                         11) ...
      |                                     );
      | if sm_RFA_RSSI_Buffer_sel_value == xfix({xlUnsigned, ...
      |                                         xl_nbits(linearAddr) - 11, ...
      |                                         0}, ...
      |                                         67);
      |     sm_RFA_RSSI_Buffer_sel = true;
      | else
      |     sm_RFA_RSSI_Buffer_sel = false;
      | end
      | sm_RFA_IQ_Rx_Buffer_sel_value = xl_concat(xl_slice(linearAddr, ...
      |                                         xl_nbits(linearAddr) - 1, ...
      |                                         14) ...
      |                                     );
      | if sm_RFA_IQ_Rx_Buffer_sel_value == xfix({xlUnsigned, ...
      |                                         xl_nbits(linearAddr) - 14, ...
      |                                         0}, ...
      |                                         7);
      |     sm_RFA_IQ_Rx_Buffer_sel = true;
      | else
      |     sm_RFA_IQ_Rx_Buffer_sel = false;
      | end
      | 
      | 
      | % registered Shared Memory mux output
      | persistent ram_bank_out_reg; ram_bank_out_reg = xl_state(0, {xlUnsigned, 32, 0});
      | ram_bank_out = ram_bank_out_reg;
      | if sm_RFD_IQ_Tx_Buffer_sel
      |     ram_bank_out_reg = sm_RFD_IQ_Tx_Buffer_bus;
      | elseif sm_RFD_RSSI_Buffer_sel
      |     ram_bank_out_reg = sm_RFD_RSSI_Buffer_bus;
      | elseif sm_RFD_IQ_Rx_Buffer_sel
      |     ram_bank_out_reg = sm_RFD_IQ_Rx_Buffer_bus;
      | elseif sm_RFC_IQ_Tx_Buffer_sel
      |     ram_bank_out_reg = sm_RFC_IQ_Tx_Buffer_bus;
      | elseif sm_RFC_RSSI_Buffer_sel
      |     ram_bank_out_reg = sm_RFC_RSSI_Buffer_bus;
      | elseif sm_RFC_IQ_Rx_Buffer_sel
      |     ram_bank_out_reg = sm_RFC_IQ_Rx_Buffer_bus;
      | elseif sm_RFB_IQ_Tx_Buffer_sel
      |     ram_bank_out_reg = sm_RFB_IQ_Tx_Buffer_bus;
      | elseif sm_RFB_RSSI_Buffer_sel
      |     ram_bank_out_reg = sm_RFB_RSSI_Buffer_bus;
      | elseif sm_RFB_IQ_Rx_Buffer_sel
      |     ram_bank_out_reg = sm_RFB_IQ_Rx_Buffer_bus;
      | elseif sm_RFA_IQ_Tx_Buffer_sel
      |     ram_bank_out_reg = sm_RFA_IQ_Tx_Buffer_bus;
      | elseif sm_RFA_RSSI_Buffer_sel
      |     ram_bank_out_reg = sm_RFA_RSSI_Buffer_bus;
      | elseif sm_RFA_IQ_Rx_Buffer_sel
      |     ram_bank_out_reg = sm_RFA_IQ_Rx_Buffer_bus;
      | end
      | 
      | % 'din' ports of 'Shared Memory' blocks
      | sm_RFD_IQ_Tx_Buffer_din = xl_force(xl_slice(wrDBus, 32 - 1, 0), ...
      |                                  xlUnsigned, ...
      |                                  0);
      | sm_RFD_RSSI_Buffer_din = xl_force(xl_slice(wrDBus, 32 - 1, 0), ...
      |                                  xlUnsigned, ...
      |                                  0);
      | sm_RFD_IQ_Rx_Buffer_din = xl_force(xl_slice(wrDBus, 32 - 1, 0), ...
      |                                  xlUnsigned, ...
      |                                  0);
      | sm_RFC_IQ_Tx_Buffer_din = xl_force(xl_slice(wrDBus, 32 - 1, 0), ...
      |                                  xlUnsigned, ...
      |                                  0);
      | sm_RFC_RSSI_Buffer_din = xl_force(xl_slice(wrDBus, 32 - 1, 0), ...
      |                                  xlUnsigned, ...
      |                                  0);
      | sm_RFC_IQ_Rx_Buffer_din = xl_force(xl_slice(wrDBus, 32 - 1, 0), ...
      |                                  xlUnsigned, ...
      |                                  0);
      | sm_RFB_IQ_Tx_Buffer_din = xl_force(xl_slice(wrDBus, 32 - 1, 0), ...
      |                                  xlUnsigned, ...
      |                                  0);
      | sm_RFB_RSSI_Buffer_din = xl_force(xl_slice(wrDBus, 32 - 1, 0), ...
      |                                  xlUnsigned, ...
      |                                  0);
      | sm_RFB_IQ_Rx_Buffer_din = xl_force(xl_slice(wrDBus, 32 - 1, 0), ...
      |                                  xlUnsigned, ...
      |                                  0);
      | sm_RFA_IQ_Tx_Buffer_din = xl_force(xl_slice(wrDBus, 32 - 1, 0), ...
      |                                  xlUnsigned, ...
      |                                  0);
      | sm_RFA_RSSI_Buffer_din = xl_force(xl_slice(wrDBus, 32 - 1, 0), ...
      |                                  xlUnsigned, ...
      |                                  0);
      | sm_RFA_IQ_Rx_Buffer_din = xl_force(xl_slice(wrDBus, 32 - 1, 0), ...
      |                                  xlUnsigned, ...
      |                                  0);
      | 
      | 
      | % 'we' ports of 'Shared Memory' blocks
      | persistent sm_RFD_IQ_Tx_Buffer_we_reg; sm_RFD_IQ_Tx_Buffer_we_reg = xl_state(false, {xlBoolean});
      | sm_RFD_IQ_Tx_Buffer_we = sm_RFD_IQ_Tx_Buffer_we_reg;
      | opCode_sm_RFD_IQ_Tx_Buffer = xl_concat(addrAck, ...
      |                                      RNWReg, ...
      |                                      bankAddr, ...
      |                                      xl_slice(linearAddr, ...
      |                                               xl_nbits(linearAddr) - 1, ...
      |                                               14) ...
      |                                     );
      | if opCode_sm_RFD_IQ_Tx_Buffer == xl_concat(xfix({xlUnsigned, 4, 0}, 8), ...
      |                                          xfix({xlUnsigned, ...
      |                                                xl_nbits(linearAddr) - 14, ...
      |                                                0}, ...
      |                                                0) ...
      |                                         );
      |     sm_RFD_IQ_Tx_Buffer_we_reg = true;
      | else
      |     sm_RFD_IQ_Tx_Buffer_we_reg = false;
      | end
      | persistent sm_RFD_RSSI_Buffer_we_reg; sm_RFD_RSSI_Buffer_we_reg = xl_state(false, {xlBoolean});
      | sm_RFD_RSSI_Buffer_we = sm_RFD_RSSI_Buffer_we_reg;
      | opCode_sm_RFD_RSSI_Buffer = xl_concat(addrAck, ...
      |                                      RNWReg, ...
      |                                      bankAddr, ...
      |                                      xl_slice(linearAddr, ...
      |                                               xl_nbits(linearAddr) - 1, ...
      |                                               11) ...
      |                                     );
      | if opCode_sm_RFD_RSSI_Buffer == xl_concat(xfix({xlUnsigned, 4, 0}, 8), ...
      |                                          xfix({xlUnsigned, ...
      |                                                xl_nbits(linearAddr) - 11, ...
      |                                                0}, ...
      |                                                64) ...
      |                                         );
      |     sm_RFD_RSSI_Buffer_we_reg = true;
      | else
      |     sm_RFD_RSSI_Buffer_we_reg = false;
      | end
      | persistent sm_RFD_IQ_Rx_Buffer_we_reg; sm_RFD_IQ_Rx_Buffer_we_reg = xl_state(false, {xlBoolean});
      | sm_RFD_IQ_Rx_Buffer_we = sm_RFD_IQ_Rx_Buffer_we_reg;
      | opCode_sm_RFD_IQ_Rx_Buffer = xl_concat(addrAck, ...
      |                                      RNWReg, ...
      |                                      bankAddr, ...
      |                                      xl_slice(linearAddr, ...
      |                                               xl_nbits(linearAddr) - 1, ...
      |                                               14) ...
      |                                     );
      | if opCode_sm_RFD_IQ_Rx_Buffer == xl_concat(xfix({xlUnsigned, 4, 0}, 8), ...
      |                                          xfix({xlUnsigned, ...
      |                                                xl_nbits(linearAddr) - 14, ...
      |                                                0}, ...
      |                                                1) ...
      |                                         );
      |     sm_RFD_IQ_Rx_Buffer_we_reg = true;
      | else
      |     sm_RFD_IQ_Rx_Buffer_we_reg = false;
      | end
      | persistent sm_RFC_IQ_Tx_Buffer_we_reg; sm_RFC_IQ_Tx_Buffer_we_reg = xl_state(false, {xlBoolean});
      | sm_RFC_IQ_Tx_Buffer_we = sm_RFC_IQ_Tx_Buffer_we_reg;
      | opCode_sm_RFC_IQ_Tx_Buffer = xl_concat(addrAck, ...
      |                                      RNWReg, ...
      |                                      bankAddr, ...
      |                                      xl_slice(linearAddr, ...
      |                                               xl_nbits(linearAddr) - 1, ...
      |                                               14) ...
      |                                     );
      | if opCode_sm_RFC_IQ_Tx_Buffer == xl_concat(xfix({xlUnsigned, 4, 0}, 8), ...
      |                                          xfix({xlUnsigned, ...
      |                                                xl_nbits(linearAddr) - 14, ...
      |                                                0}, ...
      |                                                2) ...
      |                                         );
      |     sm_RFC_IQ_Tx_Buffer_we_reg = true;
      | else
      |     sm_RFC_IQ_Tx_Buffer_we_reg = false;
      | end
      | persistent sm_RFC_RSSI_Buffer_we_reg; sm_RFC_RSSI_Buffer_we_reg = xl_state(false, {xlBoolean});
      | sm_RFC_RSSI_Buffer_we = sm_RFC_RSSI_Buffer_we_reg;
      | opCode_sm_RFC_RSSI_Buffer = xl_concat(addrAck, ...
      |                                      RNWReg, ...
      |                                      bankAddr, ...
      |                                      xl_slice(linearAddr, ...
      |                                               xl_nbits(linearAddr) - 1, ...
      |                                               11) ...
      |                                     );
      | if opCode_sm_RFC_RSSI_Buffer == xl_concat(xfix({xlUnsigned, 4, 0}, 8), ...
      |                                          xfix({xlUnsigned, ...
      |                                                xl_nbits(linearAddr) - 11, ...
      |                                                0}, ...
      |                                                65) ...
      |                                         );
      |     sm_RFC_RSSI_Buffer_we_reg = true;
      | else
      |     sm_RFC_RSSI_Buffer_we_reg = false;
      | end
      | persistent sm_RFC_IQ_Rx_Buffer_we_reg; sm_RFC_IQ_Rx_Buffer_we_reg = xl_state(false, {xlBoolean});
      | sm_RFC_IQ_Rx_Buffer_we = sm_RFC_IQ_Rx_Buffer_we_reg;
      | opCode_sm_RFC_IQ_Rx_Buffer = xl_concat(addrAck, ...
      |                                      RNWReg, ...
      |                                      bankAddr, ...
      |                                      xl_slice(linearAddr, ...
      |                                               xl_nbits(linearAddr) - 1, ...
      |                                               14) ...
      |                                     );
      | if opCode_sm_RFC_IQ_Rx_Buffer == xl_concat(xfix({xlUnsigned, 4, 0}, 8), ...
      |                                          xfix({xlUnsigned, ...
      |                                                xl_nbits(linearAddr) - 14, ...
      |                                                0}, ...
      |                                                3) ...
      |                                         );
      |     sm_RFC_IQ_Rx_Buffer_we_reg = true;
      | else
      |     sm_RFC_IQ_Rx_Buffer_we_reg = false;
      | end
      | persistent sm_RFB_IQ_Tx_Buffer_we_reg; sm_RFB_IQ_Tx_Buffer_we_reg = xl_state(false, {xlBoolean});
      | sm_RFB_IQ_Tx_Buffer_we = sm_RFB_IQ_Tx_Buffer_we_reg;
      | opCode_sm_RFB_IQ_Tx_Buffer = xl_concat(addrAck, ...
      |                                      RNWReg, ...
      |                                      bankAddr, ...
      |                                      xl_slice(linearAddr, ...
      |                                               xl_nbits(linearAddr) - 1, ...
      |                                               14) ...
      |                                     );
      | if opCode_sm_RFB_IQ_Tx_Buffer == xl_concat(xfix({xlUnsigned, 4, 0}, 8), ...
      |                                          xfix({xlUnsigned, ...
      |                                                xl_nbits(linearAddr) - 14, ...
      |                                                0}, ...
      |                                                4) ...
      |                                         );
      |     sm_RFB_IQ_Tx_Buffer_we_reg = true;
      | else
      |     sm_RFB_IQ_Tx_Buffer_we_reg = false;
      | end
      | persistent sm_RFB_RSSI_Buffer_we_reg; sm_RFB_RSSI_Buffer_we_reg = xl_state(false, {xlBoolean});
      | sm_RFB_RSSI_Buffer_we = sm_RFB_RSSI_Buffer_we_reg;
      | opCode_sm_RFB_RSSI_Buffer = xl_concat(addrAck, ...
      |                                      RNWReg, ...
      |                                      bankAddr, ...
      |                                      xl_slice(linearAddr, ...
      |                                               xl_nbits(linearAddr) - 1, ...
      |                                               11) ...
      |                                     );
      | if opCode_sm_RFB_RSSI_Buffer == xl_concat(xfix({xlUnsigned, 4, 0}, 8), ...
      |                                          xfix({xlUnsigned, ...
      |                                                xl_nbits(linearAddr) - 11, ...
      |                                                0}, ...
      |                                                66) ...
      |                                         );
      |     sm_RFB_RSSI_Buffer_we_reg = true;
      | else
      |     sm_RFB_RSSI_Buffer_we_reg = false;
      | end
      | persistent sm_RFB_IQ_Rx_Buffer_we_reg; sm_RFB_IQ_Rx_Buffer_we_reg = xl_state(false, {xlBoolean});
      | sm_RFB_IQ_Rx_Buffer_we = sm_RFB_IQ_Rx_Buffer_we_reg;
      | opCode_sm_RFB_IQ_Rx_Buffer = xl_concat(addrAck, ...
      |                                      RNWReg, ...
      |                                      bankAddr, ...
      |                                      xl_slice(linearAddr, ...
      |                                               xl_nbits(linearAddr) - 1, ...
      |                                               14) ...
      |                                     );
      | if opCode_sm_RFB_IQ_Rx_Buffer == xl_concat(xfix({xlUnsigned, 4, 0}, 8), ...
      |                                          xfix({xlUnsigned, ...
      |                                                xl_nbits(linearAddr) - 14, ...
      |                                                0}, ...
      |                                                5) ...
      |                                         );
      |     sm_RFB_IQ_Rx_Buffer_we_reg = true;
      | else
      |     sm_RFB_IQ_Rx_Buffer_we_reg = false;
      | end
      | persistent sm_RFA_IQ_Tx_Buffer_we_reg; sm_RFA_IQ_Tx_Buffer_we_reg = xl_state(false, {xlBoolean});
      | sm_RFA_IQ_Tx_Buffer_we = sm_RFA_IQ_Tx_Buffer_we_reg;
      | opCode_sm_RFA_IQ_Tx_Buffer = xl_concat(addrAck, ...
      |                                      RNWReg, ...
      |                                      bankAddr, ...
      |                                      xl_slice(linearAddr, ...
      |                                               xl_nbits(linearAddr) - 1, ...
      |                                               14) ...
      |                                     );
      | if opCode_sm_RFA_IQ_Tx_Buffer == xl_concat(xfix({xlUnsigned, 4, 0}, 8), ...
      |                                          xfix({xlUnsigned, ...
      |                                                xl_nbits(linearAddr) - 14, ...
      |                                                0}, ...
      |                                                6) ...
      |                                         );
      |     sm_RFA_IQ_Tx_Buffer_we_reg = true;
      | else
      |     sm_RFA_IQ_Tx_Buffer_we_reg = false;
      | end
      | persistent sm_RFA_RSSI_Buffer_we_reg; sm_RFA_RSSI_Buffer_we_reg = xl_state(false, {xlBoolean});
      | sm_RFA_RSSI_Buffer_we = sm_RFA_RSSI_Buffer_we_reg;
      | opCode_sm_RFA_RSSI_Buffer = xl_concat(addrAck, ...
      |                                      RNWReg, ...
      |                                      bankAddr, ...
      |                                      xl_slice(linearAddr, ...
      |                                               xl_nbits(linearAddr) - 1, ...
      |                                               11) ...
      |                                     );
      | if opCode_sm_RFA_RSSI_Buffer == xl_concat(xfix({xlUnsigned, 4, 0}, 8), ...
      |                                          xfix({xlUnsigned, ...
      |                                                xl_nbits(linearAddr) - 11, ...
      |                                                0}, ...
      |                                                67) ...
      |                                         );
      |     sm_RFA_RSSI_Buffer_we_reg = true;
      | else
      |     sm_RFA_RSSI_Buffer_we_reg = false;
      | end
      | persistent sm_RFA_IQ_Rx_Buffer_we_reg; sm_RFA_IQ_Rx_Buffer_we_reg = xl_state(false, {xlBoolean});
      | sm_RFA_IQ_Rx_Buffer_we = sm_RFA_IQ_Rx_Buffer_we_reg;
      | opCode_sm_RFA_IQ_Rx_Buffer = xl_concat(addrAck, ...
      |                                      RNWReg, ...
      |                                      bankAddr, ...
      |                                      xl_slice(linearAddr, ...
      |                                               xl_nbits(linearAddr) - 1, ...
      |                                               14) ...
      |                                     );
      | if opCode_sm_RFA_IQ_Rx_Buffer == xl_concat(xfix({xlUnsigned, 4, 0}, 8), ...
      |                                          xfix({xlUnsigned, ...
      |                                                xl_nbits(linearAddr) - 14, ...
      |                                                0}, ...
      |                                                7) ...
      |                                         );
      |     sm_RFA_IQ_Rx_Buffer_we_reg = true;
      | else
      |     sm_RFA_IQ_Rx_Buffer_we_reg = false;
      | end
      | 
      | 
      | % 'addr' ports of 'Shared Memory' blocks
      | persistent sm_RFD_IQ_Tx_Buffer_addr_reg; 
      | sm_RFD_IQ_Tx_Buffer_addr_reg = xl_state(0, {xlUnsigned, 14, 0});
      | sm_RFD_IQ_Tx_Buffer_addr = sm_RFD_IQ_Tx_Buffer_addr_reg;
      | if addrAck == 1
      |     sm_RFD_IQ_Tx_Buffer_addr_reg = xl_slice(linearAddr, 14, 0);
      | else
      |     sm_RFD_IQ_Tx_Buffer_addr_reg = sm_RFD_IQ_Tx_Buffer_addr_reg;
      | end
      | persistent sm_RFD_RSSI_Buffer_addr_reg; 
      | sm_RFD_RSSI_Buffer_addr_reg = xl_state(0, {xlUnsigned, 11, 0});
      | sm_RFD_RSSI_Buffer_addr = sm_RFD_RSSI_Buffer_addr_reg;
      | if addrAck == 1
      |     sm_RFD_RSSI_Buffer_addr_reg = xl_slice(linearAddr, 11, 0);
      | else
      |     sm_RFD_RSSI_Buffer_addr_reg = sm_RFD_RSSI_Buffer_addr_reg;
      | end
      | persistent sm_RFD_IQ_Rx_Buffer_addr_reg; 
      | sm_RFD_IQ_Rx_Buffer_addr_reg = xl_state(0, {xlUnsigned, 14, 0});
      | sm_RFD_IQ_Rx_Buffer_addr = sm_RFD_IQ_Rx_Buffer_addr_reg;
      | if addrAck == 1
      |     sm_RFD_IQ_Rx_Buffer_addr_reg = xl_slice(linearAddr, 14, 0);
      | else
      |     sm_RFD_IQ_Rx_Buffer_addr_reg = sm_RFD_IQ_Rx_Buffer_addr_reg;
      | end
      | persistent sm_RFC_IQ_Tx_Buffer_addr_reg; 
      | sm_RFC_IQ_Tx_Buffer_addr_reg = xl_state(0, {xlUnsigned, 14, 0});
      | sm_RFC_IQ_Tx_Buffer_addr = sm_RFC_IQ_Tx_Buffer_addr_reg;
      | if addrAck == 1
      |     sm_RFC_IQ_Tx_Buffer_addr_reg = xl_slice(linearAddr, 14, 0);
      | else
      |     sm_RFC_IQ_Tx_Buffer_addr_reg = sm_RFC_IQ_Tx_Buffer_addr_reg;
      | end
      | persistent sm_RFC_RSSI_Buffer_addr_reg; 
      | sm_RFC_RSSI_Buffer_addr_reg = xl_state(0, {xlUnsigned, 11, 0});
      | sm_RFC_RSSI_Buffer_addr = sm_RFC_RSSI_Buffer_addr_reg;
      | if addrAck == 1
      |     sm_RFC_RSSI_Buffer_addr_reg = xl_slice(linearAddr, 11, 0);
      | else
      |     sm_RFC_RSSI_Buffer_addr_reg = sm_RFC_RSSI_Buffer_addr_reg;
      | end
      | persistent sm_RFC_IQ_Rx_Buffer_addr_reg; 
      | sm_RFC_IQ_Rx_Buffer_addr_reg = xl_state(0, {xlUnsigned, 14, 0});
      | sm_RFC_IQ_Rx_Buffer_addr = sm_RFC_IQ_Rx_Buffer_addr_reg;
      | if addrAck == 1
      |     sm_RFC_IQ_Rx_Buffer_addr_reg = xl_slice(linearAddr, 14, 0);
      | else
      |     sm_RFC_IQ_Rx_Buffer_addr_reg = sm_RFC_IQ_Rx_Buffer_addr_reg;
      | end
      | persistent sm_RFB_IQ_Tx_Buffer_addr_reg; 
      | sm_RFB_IQ_Tx_Buffer_addr_reg = xl_state(0, {xlUnsigned, 14, 0});
      | sm_RFB_IQ_Tx_Buffer_addr = sm_RFB_IQ_Tx_Buffer_addr_reg;
      | if addrAck == 1
      |     sm_RFB_IQ_Tx_Buffer_addr_reg = xl_slice(linearAddr, 14, 0);
      | else
      |     sm_RFB_IQ_Tx_Buffer_addr_reg = sm_RFB_IQ_Tx_Buffer_addr_reg;
      | end
      | persistent sm_RFB_RSSI_Buffer_addr_reg; 
      | sm_RFB_RSSI_Buffer_addr_reg = xl_state(0, {xlUnsigned, 11, 0});
      | sm_RFB_RSSI_Buffer_addr = sm_RFB_RSSI_Buffer_addr_reg;
      | if addrAck == 1
      |     sm_RFB_RSSI_Buffer_addr_reg = xl_slice(linearAddr, 11, 0);
      | else
      |     sm_RFB_RSSI_Buffer_addr_reg = sm_RFB_RSSI_Buffer_addr_reg;
      | end
      | persistent sm_RFB_IQ_Rx_Buffer_addr_reg; 
      | sm_RFB_IQ_Rx_Buffer_addr_reg = xl_state(0, {xlUnsigned, 14, 0});
      | sm_RFB_IQ_Rx_Buffer_addr = sm_RFB_IQ_Rx_Buffer_addr_reg;
      | if addrAck == 1
      |     sm_RFB_IQ_Rx_Buffer_addr_reg = xl_slice(linearAddr, 14, 0);
      | else
      |     sm_RFB_IQ_Rx_Buffer_addr_reg = sm_RFB_IQ_Rx_Buffer_addr_reg;
      | end
      | persistent sm_RFA_IQ_Tx_Buffer_addr_reg; 
      | sm_RFA_IQ_Tx_Buffer_addr_reg = xl_state(0, {xlUnsigned, 14, 0});
      | sm_RFA_IQ_Tx_Buffer_addr = sm_RFA_IQ_Tx_Buffer_addr_reg;
      | if addrAck == 1
      |     sm_RFA_IQ_Tx_Buffer_addr_reg = xl_slice(linearAddr, 14, 0);
      | else
      |     sm_RFA_IQ_Tx_Buffer_addr_reg = sm_RFA_IQ_Tx_Buffer_addr_reg;
      | end
      | persistent sm_RFA_RSSI_Buffer_addr_reg; 
      | sm_RFA_RSSI_Buffer_addr_reg = xl_state(0, {xlUnsigned, 11, 0});
      | sm_RFA_RSSI_Buffer_addr = sm_RFA_RSSI_Buffer_addr_reg;
      | if addrAck == 1
      |     sm_RFA_RSSI_Buffer_addr_reg = xl_slice(linearAddr, 11, 0);
      | else
      |     sm_RFA_RSSI_Buffer_addr_reg = sm_RFA_RSSI_Buffer_addr_reg;
      | end
      | persistent sm_RFA_IQ_Rx_Buffer_addr_reg; 
      | sm_RFA_IQ_Rx_Buffer_addr_reg = xl_state(0, {xlUnsigned, 14, 0});
      | sm_RFA_IQ_Rx_Buffer_addr = sm_RFA_IQ_Rx_Buffer_addr_reg;
      | if addrAck == 1
      |     sm_RFA_IQ_Rx_Buffer_addr_reg = xl_slice(linearAddr, 14, 0);
      | else
      |     sm_RFA_IQ_Rx_Buffer_addr_reg = sm_RFA_IQ_Rx_Buffer_addr_reg;
      | end
      | 
      | 
      | % 're' ports of 'From FIFO' blocks
      | 
      | 
      | % 'en' ports of 'To Register' blocks
      | if opCode == xl_concat(xfix({xlUnsigned, 4, 0}, 10), ...
      |                        xfix({xlUnsigned, xl_nbits(linearAddr), 0}, 0))
      |     sm_TX_DELAY_en = true;
      | else
      |     sm_TX_DELAY_en = false;
      | end
      | if opCode == xl_concat(xfix({xlUnsigned, 4, 0}, 10), ...
      |                        xfix({xlUnsigned, xl_nbits(linearAddr), 0}, 1))
      |     sm_RF_RX_IQ_BUF_RD_BYTE_OFFSET_en = true;
      | else
      |     sm_RF_RX_IQ_BUF_RD_BYTE_OFFSET_en = false;
      | end
      | if opCode == xl_concat(xfix({xlUnsigned, 4, 0}, 10), ...
      |                        xfix({xlUnsigned, xl_nbits(linearAddr), 0}, 2))
      |     sm_LOAD_TIMER_64_LSB_en = true;
      | else
      |     sm_LOAD_TIMER_64_LSB_en = false;
      | end
      | if opCode == xl_concat(xfix({xlUnsigned, 4, 0}, 10), ...
      |                        xfix({xlUnsigned, xl_nbits(linearAddr), 0}, 3))
      |     sm_RF_RX_IQ_THRESHOLD_en = true;
      | else
      |     sm_RF_RX_IQ_THRESHOLD_en = false;
      | end
      | if opCode == xl_concat(xfix({xlUnsigned, 4, 0}, 10), ...
      |                        xfix({xlUnsigned, xl_nbits(linearAddr), 0}, 4))
      |     sm_RX_LENGTH_en = true;
      | else
      |     sm_RX_LENGTH_en = false;
      | end
      | if opCode == xl_concat(xfix({xlUnsigned, 4, 0}, 10), ...
      |                        xfix({xlUnsigned, xl_nbits(linearAddr), 0}, 5))
      |     sm_TX_LENGTH_en = true;
      | else
      |     sm_TX_LENGTH_en = false;
      | end
      | if opCode == xl_concat(xfix({xlUnsigned, 4, 0}, 10), ...
      |                        xfix({xlUnsigned, xl_nbits(linearAddr), 0}, 6))
      |     sm_RF_RX_IQ_BUF_WR_BYTE_OFFSET_en = true;
      | else
      |     sm_RF_RX_IQ_BUF_WR_BYTE_OFFSET_en = false;
      | end
      | if opCode == xl_concat(xfix({xlUnsigned, 4, 0}, 10), ...
      |                        xfix({xlUnsigned, xl_nbits(linearAddr), 0}, 7))
      |     sm_RF_BUFFER_SEL_en = true;
      | else
      |     sm_RF_BUFFER_SEL_en = false;
      | end
      | if opCode == xl_concat(xfix({xlUnsigned, 4, 0}, 10), ...
      |                        xfix({xlUnsigned, xl_nbits(linearAddr), 0}, 8))
      |     sm_RX_BUF_EN_en = true;
      | else
      |     sm_RX_BUF_EN_en = false;
      | end
      | if opCode == xl_concat(xfix({xlUnsigned, 4, 0}, 10), ...
      |                        xfix({xlUnsigned, xl_nbits(linearAddr), 0}, 9))
      |     sm_RF_TX_IQ_THRESHOLD_en = true;
      | else
      |     sm_RF_TX_IQ_THRESHOLD_en = false;
      | end
      | if opCode == xl_concat(xfix({xlUnsigned, 4, 0}, 10), ...
      |                        xfix({xlUnsigned, xl_nbits(linearAddr), 0}, 10))
      |     sm_CONFIG_en = true;
      | else
      |     sm_CONFIG_en = false;
      | end
      | if opCode == xl_concat(xfix({xlUnsigned, 4, 0}, 10), ...
      |                        xfix({xlUnsigned, xl_nbits(linearAddr), 0}, 11))
      |     sm_RF_ERROR_CLR_en = true;
      | else
      |     sm_RF_ERROR_CLR_en = false;
      | end
      | if opCode == xl_concat(xfix({xlUnsigned, 4, 0}, 10), ...
      |                        xfix({xlUnsigned, xl_nbits(linearAddr), 0}, 12))
      |     sm_RF_TX_IQ_BUF_WR_BYTE_OFFSET_en = true;
      | else
      |     sm_RF_TX_IQ_BUF_WR_BYTE_OFFSET_en = false;
      | end
      | if opCode == xl_concat(xfix({xlUnsigned, 4, 0}, 10), ...
      |                        xfix({xlUnsigned, xl_nbits(linearAddr), 0}, 13))
      |     sm_LOAD_TIMER_64_MSB_en = true;
      | else
      |     sm_LOAD_TIMER_64_MSB_en = false;
      | end
      | if opCode == xl_concat(xfix({xlUnsigned, 4, 0}, 10), ...
      |                        xfix({xlUnsigned, xl_nbits(linearAddr), 0}, 14))
      |     sm_TX_BUF_EN_en = true;
      | else
      |     sm_TX_BUF_EN_en = false;
      | end
      | 
      | 
      | % 'din' ports of 'To FIFO' blocks
      | 
      | 
      | % 'we' ports of 'To FIFO' blocks
      | 
      | 
      | % 'din' ports of 'To Register' blocks
      | sm_TX_DELAY_din = xl_force(xl_slice(wrDBus, 32 - 1, 0), ...
      |                                  xlUnsigned, ...
      |                                  0);
      | sm_RF_RX_IQ_BUF_RD_BYTE_OFFSET_din = xl_force(xl_slice(wrDBus, 32 - 1, 0), ...
      |                                  xlUnsigned, ...
      |                                  0);
      | sm_LOAD_TIMER_64_LSB_din = xl_force(xl_slice(wrDBus, 32 - 1, 0), ...
      |                                  xlUnsigned, ...
      |                                  0);
      | sm_RF_RX_IQ_THRESHOLD_din = xl_force(xl_slice(wrDBus, 32 - 1, 0), ...
      |                                  xlUnsigned, ...
      |                                  0);
      | sm_RX_LENGTH_din = xl_force(xl_slice(wrDBus, 32 - 1, 0), ...
      |                                  xlUnsigned, ...
      |                                  0);
      | sm_TX_LENGTH_din = xl_force(xl_slice(wrDBus, 32 - 1, 0), ...
      |                                  xlUnsigned, ...
      |                                  0);
      | sm_RF_RX_IQ_BUF_WR_BYTE_OFFSET_din = xl_force(xl_slice(wrDBus, 32 - 1, 0), ...
      |                                  xlUnsigned, ...
      |                                  0);
      | sm_RF_BUFFER_SEL_din = xl_force(xl_slice(wrDBus, 32 - 1, 0), ...
      |                                  xlUnsigned, ...
      |                                  0);
      | sm_RX_BUF_EN_din = xl_force(xl_slice(wrDBus, 32 - 1, 0), ...
      |                                  xlUnsigned, ...
      |                                  0);
      | sm_RF_TX_IQ_THRESHOLD_din = xl_force(xl_slice(wrDBus, 32 - 1, 0), ...
      |                                  xlUnsigned, ...
      |                                  0);
      | sm_CONFIG_din = xl_force(xl_slice(wrDBus, 32 - 1, 0), ...
      |                                  xlUnsigned, ...
      |                                  0);
      | sm_RF_ERROR_CLR_din = xl_force(xl_slice(wrDBus, 9 - 1, 0), ...
      |                                  xlUnsigned, ...
      |                                  0);
      | sm_RF_TX_IQ_BUF_WR_BYTE_OFFSET_din = xl_force(xl_slice(wrDBus, 32 - 1, 0), ...
      |                                  xlUnsigned, ...
      |                                  0);
      | sm_LOAD_TIMER_64_MSB_din = xl_force(xl_slice(wrDBus, 32 - 1, 0), ...
      |                                  xlUnsigned, ...
      |                                  0);
      | sm_TX_BUF_EN_din = xl_force(xl_slice(wrDBus, 32 - 1, 0), ...
      |                                  xlUnsigned, ...
      |                                  0);
      | 
      | 
      | persistent read_bank_out_reg; read_bank_out_reg = xl_state(0, {xlUnsigned, 32, 0});
      | read_bank_out = read_bank_out_reg;
      | 
      | persistent bankAddr_reg; bankAddr_reg = xl_state(0, bankAddr);
      | 
      | if bankAddr_reg == 0
      |     % Bank 0: Shared Memories
      |     read_bank_out_reg = ram_bank_out;
      | elseif bankAddr_reg == 1
      |     % Bank 1: From/To FIFOs
      |     read_bank_out_reg =  0;
      | elseif bankAddr_reg == 2
      |     % Bank 2: From/To Registers
      |     read_bank_out_reg = reg_bank_out;
      | elseif bankAddr_reg == 3
      |     % Bank 3: Configuration Registers
      |     read_bank_out_reg = 0;
      | end
      | 
      | bankAddr_reg = bankAddr;
  sg_plb_addrpref : xbsIndex_r4/Gateway In  gui_display_data_type=Fixed-point  arith_type=Unsigned  n_bits=10  bin_pt=0  preci_type=Single  exp_width=8  frac_width=24  quantization="Round  (unbiased: +/- Inf)"  overflow=Saturate  period=xlGetNormalizedPeriod()  dbl_ovrd=off  timing_constraint=None  locs_specified=off  LOCs={}  UseAsADC=off  ADCChannel='1'  inherit_from_input=off  hdl_port=on  block_type=gatewayin
      settings: sginterface={'Xilinx'=>{'jtaghwcosim'=>{'non_memory_mapped_port'=>'sg_plb_addrpref'}},'iopad'=>{'constraint'=>'#'}}
  wires:
  plb_decode/2 -> plb_memmap/5, Sl_addrAck/1  "Sl_addrAck"
  plb_decode/4 -> Sl_wrDAck/1, Sl_wrComp/1  "Sl_wrDAck"
  plb_memmap/67 -> Shared Memory11/3  "RFA_IQ_Rx_Buffer_we"
  plb_memmap/66 -> Shared Memory11/2  "RFA_IQ_Rx_Buffer_din"
  plb_memmap/65 -> Shared Memory11/1  "RFA_IQ_Rx_Buffer_addr"
  plb_memmap/64 -> Shared Memory10/3  "RFA_RSSI_Buffer_we"
  plb_memmap/63 -> Shared Memory10/2  "RFA_RSSI_Buffer_din"
  plb_memmap/62 -> Shared Memory10/1  "RFA_RSSI_Buffer_addr"
  plb_memmap/61 -> Shared Memory9/3  "RFA_IQ_Tx_Buffer_we"
  plb_memmap/60 -> Shared Memory9/2  "RFA_IQ_Tx_Buffer_din"
  plb_memmap/59 -> Shared Memory9/1  "RFA_IQ_Tx_Buffer_addr"
  plb_memmap/58 -> Shared Memory8/3  "RFB_IQ_Rx_Buffer_we"
  plb_memmap/57 -> Shared Memory8/2  "RFB_IQ_Rx_Buffer_din"
  plb_memmap/56 -> Shared Memory8/1  "RFB_IQ_Rx_Buffer_addr"
  plb_memmap/55 -> Shared Memory7/3  "RFB_RSSI_Buffer_we"
  plb_memmap/54 -> Shared Memory7/2  "RFB_RSSI_Buffer_din"
  plb_memmap/53 -> Shared Memory7/1  "RFB_RSSI_Buffer_addr"
  plb_memmap/52 -> Shared Memory6/3  "RFB_IQ_Tx_Buffer_we"
  plb_memmap/51 -> Shared Memory6/2  "RFB_IQ_Tx_Buffer_din"
  plb_memmap/50 -> Shared Memory6/1  "RFB_IQ_Tx_Buffer_addr"
  plb_memmap/49 -> Shared Memory5/3  "RFC_IQ_Rx_Buffer_we"
  plb_memmap/48 -> Shared Memory5/2  "RFC_IQ_Rx_Buffer_din"
  plb_memmap/47 -> Shared Memory5/1  "RFC_IQ_Rx_Buffer_addr"
  plb_memmap/46 -> Shared Memory4/3  "RFC_RSSI_Buffer_we"
  plb_memmap/45 -> Shared Memory4/2  "RFC_RSSI_Buffer_din"
  plb_memmap/44 -> Shared Memory4/1  "RFC_RSSI_Buffer_addr"
  plb_memmap/43 -> Shared Memory3/3  "RFC_IQ_Tx_Buffer_we"
  plb_memmap/42 -> Shared Memory3/2  "RFC_IQ_Tx_Buffer_din"
  plb_memmap/41 -> Shared Memory3/1  "RFC_IQ_Tx_Buffer_addr"
  plb_memmap/40 -> Shared Memory2/3  "RFD_IQ_Rx_Buffer_we"
  plb_memmap/39 -> Shared Memory2/2  "RFD_IQ_Rx_Buffer_din"
  plb_memmap/38 -> Shared Memory2/1  "RFD_IQ_Rx_Buffer_addr"
  plb_memmap/37 -> Shared Memory1/3  "RFD_RSSI_Buffer_we"
  plb_memmap/36 -> Shared Memory1/2  "RFD_RSSI_Buffer_din"
  plb_memmap/35 -> Shared Memory1/1  "RFD_RSSI_Buffer_addr"
  plb_memmap/34 -> Shared Memory/3  "RFD_IQ_Tx_Buffer_we"
  plb_memmap/33 -> Shared Memory/2  "RFD_IQ_Tx_Buffer_din"
  plb_memmap/32 -> Shared Memory/1  "RFD_IQ_Tx_Buffer_addr"
  plb_memmap/31 -> To Register14/2  "TX_BUF_EN_en"
  plb_memmap/30 -> To Register14/1  "TX_BUF_EN_din"
  plb_memmap/29 -> To Register13/2  "LOAD_TIMER_64_MSB_en"
  plb_memmap/28 -> To Register13/1  "LOAD_TIMER_64_MSB_din"
  plb_memmap/27 -> To Register12/2  "RF_TX_IQ_BUF_WR_BYTE_OFFSET_en"
  plb_memmap/26 -> To Register12/1  "RF_TX_IQ_BUF_WR_BYTE_OFFSET_din"
  plb_memmap/25 -> To Register11/2  "RF_ERROR_CLR_en"
  plb_memmap/24 -> To Register11/1  "RF_ERROR_CLR_din"
  plb_memmap/23 -> To Register10/2  "CONFIG_en"
  plb_memmap/22 -> To Register10/1  "CONFIG_din"
  plb_memmap/21 -> To Register9/2  "RF_TX_IQ_THRESHOLD_en"
  plb_memmap/20 -> To Register9/1  "RF_TX_IQ_THRESHOLD_din"
  plb_memmap/19 -> To Register8/2  "RX_BUF_EN_en"
  plb_memmap/18 -> To Register8/1  "RX_BUF_EN_din"
  plb_memmap/17 -> To Register7/2  "RF_BUFFER_SEL_en"
  plb_memmap/16 -> To Register7/1  "RF_BUFFER_SEL_din"
  plb_memmap/15 -> To Register6/2  "RF_RX_IQ_BUF_WR_BYTE_OFFSET_en"
  plb_memmap/14 -> To Register6/1  "RF_RX_IQ_BUF_WR_BYTE_OFFSET_din"
  plb_memmap/13 -> To Register5/2  "TX_LENGTH_en"
  plb_memmap/12 -> To Register5/1  "TX_LENGTH_din"
  plb_memmap/11 -> To Register4/2  "RX_LENGTH_en"
  plb_memmap/10 -> To Register4/1  "RX_LENGTH_din"
  plb_memmap/9 -> To Register3/2  "RF_RX_IQ_THRESHOLD_en"
  plb_memmap/8 -> To Register3/1  "RF_RX_IQ_THRESHOLD_din"
  plb_memmap/7 -> To Register2/2  "LOAD_TIMER_64_LSB_en"
  plb_memmap/6 -> To Register2/1  "LOAD_TIMER_64_LSB_din"
  plb_memmap/5 -> To Register1/2  "RF_RX_IQ_BUF_RD_BYTE_OFFSET_en"
  plb_memmap/4 -> To Register1/1  "RF_RX_IQ_BUF_RD_BYTE_OFFSET_din"
  plb_memmap/3 -> To Register/2  "TX_DELAY_en"
  plb_memmap/2 -> To Register/1  "TX_DELAY_din"
  plb_memmap/1 -> plb_decode/6  "rdData"
  Shared Memory11/1 -> plb_memmap/47  "RFA_IQ_Rx_Buffer_dout"
  Shared Memory10/1 -> plb_memmap/46  "RFA_RSSI_Buffer_dout"
  Shared Memory9/1 -> plb_memmap/45  "RFA_IQ_Tx_Buffer_dout"
  Shared Memory8/1 -> plb_memmap/44  "RFB_IQ_Rx_Buffer_dout"
  Shared Memory7/1 -> plb_memmap/43  "RFB_RSSI_Buffer_dout"
  Shared Memory6/1 -> plb_memmap/42  "RFB_IQ_Tx_Buffer_dout"
  Shared Memory5/1 -> plb_memmap/41  "RFC_IQ_Rx_Buffer_dout"
  Shared Memory4/1 -> plb_memmap/40  "RFC_RSSI_Buffer_dout"
  Shared Memory3/1 -> plb_memmap/39  "RFC_IQ_Tx_Buffer_dout"
  Shared Memory2/1 -> plb_memmap/38  "RFD_IQ_Rx_Buffer_dout"
  Shared Memory1/1 -> plb_memmap/37  "RFD_RSSI_Buffer_dout"
  Shared Memory/1 -> plb_memmap/36  "RFD_IQ_Tx_Buffer_dout"
  To Register14/1 -> plb_memmap/35  "TX_BUF_EN_dout"
  To Register13/1 -> plb_memmap/34  "LOAD_TIMER_64_MSB_dout"
  To Register12/1 -> plb_memmap/33  "RF_TX_IQ_BUF_WR_BYTE_OFFSET_dout"
  To Register11/1 -> plb_memmap/32  "RF_ERROR_CLR_dout"
  To Register10/1 -> plb_memmap/31  "CONFIG_dout"
  To Register9/1 -> plb_memmap/30  "RF_TX_IQ_THRESHOLD_dout"
  To Register8/1 -> plb_memmap/29  "RX_BUF_EN_dout"
  To Register7/1 -> plb_memmap/28  "RF_BUFFER_SEL_dout"
  To Register6/1 -> plb_memmap/27  "RF_RX_IQ_BUF_WR_BYTE_OFFSET_dout"
  To Register5/1 -> plb_memmap/26  "TX_LENGTH_dout"
  To Register4/1 -> plb_memmap/25  "RX_LENGTH_dout"
  To Register3/1 -> plb_memmap/24  "RF_RX_IQ_THRESHOLD_dout"
  To Register2/1 -> plb_memmap/23  "LOAD_TIMER_64_LSB_dout"
  To Register1/1 -> plb_memmap/22  "RF_RX_IQ_BUF_RD_BYTE_OFFSET_dout"
  To Register/1 -> plb_memmap/21  "TX_DELAY_dout"
  From Register14/1 -> plb_memmap/20  "AGC_DONE_ADDR_dout"
  From Register13/1 -> plb_memmap/19  "TIMER_64_LSB_dout"
  From Register12/1 -> plb_memmap/18  "TIMER_64_MSB_dout"
  From Register11/1 -> plb_memmap/17  "RFAB_AGC_DONE_RSSI_dout"
  From Register10/1 -> plb_memmap/16  "RFCD_AGC_DONE_RSSI_dout"
  From Register9/1 -> plb_memmap/15  "STATUS_dout"
  From Register8/1 -> plb_memmap/14  "RF_TX_IQ_STATUS_dout"
  From Register7/1 -> plb_memmap/13  "DESIGN_VER_dout"
  From Register6/1 -> plb_memmap/12  "BUFF_SIZES_dout"
  From Register5/1 -> plb_memmap/11  "INT_STATUS_dout"
  From Register4/1 -> plb_memmap/10  "RF_RX_IQ_BUF_WR_BYTE_OFFSET_UPDATE_dout"
  From Register3/1 -> plb_memmap/9  "RF_RX_IQ_BUF_OCCUPANCY_dout"
  From Register2/1 -> plb_memmap/8  "AGC_GAINS_dout"
  From Register1/1 -> plb_memmap/7  "RF_TX_IQ_BUF_RD_BYTE_OFFSET_dout"
  From Register/1 -> plb_memmap/6  "RF_TX_IQ_BUF_OCCUPANCY_dout"
  plb_decode/6 -> plb_memmap/4  "RNWReg"
  plb_decode/9 -> plb_memmap/3  "linearAddr"
  plb_decode/5 -> plb_memmap/2  "bankAddr"
  plb_decode/1 -> plb_memmap/1  "wrDBusReg"
  plb_decode/8 -> Sl_rdDBus/1  "Sl_rdDBus"
  plb_decode/7 -> Sl_rdDAck/1  "Sl_rdDAck"
  plb_decode/3 -> Sl_rdComp/1  "Sl_rdComp"
  sg_plb_addrpref/1 -> plb_decode/7  "addrPref"
  PLB_wrDBus/1 -> plb_decode/5  "PLB_wrDBus"
  PLB_RNW/1 -> plb_decode/4  "PLB_RNW"
  PLB_PAValid/1 -> plb_decode/3  "PLB_PAValid"
  PLB_ABus/1 -> plb_decode/2  "PLB_ABus"
  SPLB_Rst/1 -> plb_decode/1  "SPLB_Rst"
  Constant6/1 -> sg_plb_addrpref/1
  Constant5/1 -> Sl_wait/1  "Sl_wait"
  Constant4/1 -> PLB_wrDBus/1
  Constant3/1 -> PLB_RNW/1
  Constant2/1 -> PLB_PAValid/1
  Constant1/1 -> PLB_ABus/1
  Constant/1 -> SPLB_Rst/1
  Sl_wrComp/1 -> Terminator6/1
  Sl_wrDAck/1 -> Terminator5/1
  Sl_wait/1 -> Terminator4/1
  Sl_rdDBus/1 -> Terminator3/1
  Sl_rdDAck/1 -> Terminator2/1
  Sl_rdComp/1 -> Terminator1/1
  Sl_addrAck/1 -> Terminator/1
